simulink model "LKAS_AutoSave_DF_20220221_1634"  (R2018b)
(part 2 of 20)

  | T_p_kPa_1_1_u8.SlopeAdjustmentFactor = 1;
  | T_p_kPa_1_1_u8.Bias = 0;
  | T_p_kPa_1_1_u8.DataTypeOverride = 'Inherit';
  | T_p_kPa_1_1_u8.IsAlias = true;
  | 
  | T_p_kPa_256_1_u16 = Simulink.NumericType;
  | T_p_kPa_256_1_u16.Description = 'kPa (kiloPascals  (kPa))';
  | if (tmpVer > 7.11)
  | 	T_p_kPa_256_1_u16.DataScope = 'Auto';
  | end
  | T_p_kPa_256_1_u16.HeaderFile = 'Rte_Type.h';
  | T_p_kPa_256_1_u16.DataTypeMode = 'Fixed-point: slope and bias scaling';
  | T_p_kPa_256_1_u16.SignednessBool = false;
  | T_p_kPa_256_1_u16.WordLength = 16;
  | T_p_kPa_256_1_u16.FixedExponent = -8;
  | T_p_kPa_256_1_u16.SlopeAdjustmentFactor = 1;
  | T_p_kPa_256_1_u16.Bias = 0;
  | T_p_kPa_256_1_u16.DataTypeOverride = 'Inherit';
  | T_p_kPa_256_1_u16.IsAlias = true;
  | 
  | T_p_kPa_32_1_u16 = Simulink.NumericType;
  | T_p_kPa_32_1_u16.Description = 'kPa (kiloPascals  (kPa))';
  | if (tmpVer > 7.11)
  | 	T_p_kPa_32_1_u16.DataScope = 'Auto';
  | end
  | T_p_kPa_32_1_u16.HeaderFile = 'Rte_Type.h';
  | T_p_kPa_32_1_u16.DataTypeMode = 'Fixed-point: slope and bias scaling';
  | T_p_kPa_32_1_u16.SignednessBool = false;
  | T_p_kPa_32_1_u16.WordLength = 16;
  | T_p_kPa_32_1_u16.FixedExponent = -5;
  | T_p_kPa_32_1_u16.SlopeAdjustmentFactor = 1;
  | T_p_kPa_32_1_u16.Bias = 0;
  | T_p_kPa_32_1_u16.DataTypeOverride = 'Inherit';
  | T_p_kPa_32_1_u16.IsAlias = true;
  | 
  | T_p_kPa_64_1_s16 = Simulink.NumericType;
  | T_p_kPa_64_1_s16.Description = 'kPa (kiloPascals  (kPa))';
  | if (tmpVer > 7.11)
  | 	T_p_kPa_64_1_s16.DataScope = 'Auto';
  | end
  | T_p_kPa_64_1_s16.HeaderFile = 'Rte_Type.h';
  | T_p_kPa_64_1_s16.DataTypeMode = 'Fixed-point: slope and bias scaling';
  | T_p_kPa_64_1_s16.SignednessBool = true;
  | T_p_kPa_64_1_s16.WordLength = 16;
  | T_p_kPa_64_1_s16.FixedExponent = -6;
  | T_p_kPa_64_1_s16.SlopeAdjustmentFactor = 1;
  | T_p_kPa_64_1_s16.Bias = 0;
  | T_p_kPa_64_1_s16.DataTypeOverride = 'Inherit';
  | T_p_kPa_64_1_s16.IsAlias = true;
  | 
  | T_p_kPa_Float32 = Simulink.NumericType;
  | T_p_kPa_Float32.Description = 'kPa (kiloPascals  (kPa))';
  | if (tmpVer > 7.11)
  | 	T_p_kPa_Float32.DataScope = 'Auto';
  | end
  | T_p_kPa_Float32.HeaderFile = 'Rte_Type.h';
  | T_p_kPa_Float32.DataTypeMode = 'Single';
  | T_p_kPa_Float32.SignednessBool = true;
  | T_p_kPa_Float32.WordLength = 32;
  | T_p_kPa_Float32.FixedExponent = 0;
  | T_p_kPa_Float32.SlopeAdjustmentFactor = 1;
  | T_p_kPa_Float32.Bias = 0;
  | T_p_kPa_Float32.DataTypeOverride = 'Inherit';
  | T_p_kPa_Float32.IsAlias = true;
  | 
  | T_phi_deg_100_1_s16 = Simulink.NumericType;
  | T_phi_deg_100_1_s16.Description = 'deg (degrees (deg))';
  | if (tmpVer > 7.11)
  | 	T_phi_deg_100_1_s16.DataScope = 'Auto';
  | end
  | T_phi_deg_100_1_s16.HeaderFile = 'Rte_Type.h';
  | T_phi_deg_100_1_s16.DataTypeMode = ['Fixed-point: slope and bias scalin' ...
  |                                     'g'];
  | T_phi_deg_100_1_s16.SignednessBool = true;
  | T_phi_deg_100_1_s16.WordLength = 16;
  | T_phi_deg_100_1_s16.FixedExponent = -7;
  | T_phi_deg_100_1_s16.SlopeAdjustmentFactor = 1.28;
  | T_phi_deg_100_1_s16.Bias = 0;
  | T_phi_deg_100_1_s16.DataTypeOverride = 'Inherit';
  | T_phi_deg_100_1_s16.IsAlias = true;
  | 
  | T_phi_deg_1024_1_s16 = Simulink.NumericType;
  | T_phi_deg_1024_1_s16.Description = 'deg (degrees (deg))';
  | if (tmpVer > 7.11)
  | 	T_phi_deg_1024_1_s16.DataScope = 'Auto';
  | end
  | T_phi_deg_1024_1_s16.HeaderFile = 'Rte_Type.h';
  | T_phi_deg_1024_1_s16.DataTypeMode = ...
  |   'Fixed-point: slope and bias scaling';
  | T_phi_deg_1024_1_s16.SignednessBool = true;
  | T_phi_deg_1024_1_s16.WordLength = 16;
  | T_phi_deg_1024_1_s16.FixedExponent = -10;
  | T_phi_deg_1024_1_s16.SlopeAdjustmentFactor = 1;
  | T_phi_deg_1024_1_s16.Bias = 0;
  | T_phi_deg_1024_1_s16.DataTypeOverride = 'Inherit';
  | T_phi_deg_1024_1_s16.IsAlias = true;
  | 
  | T_phi_deg_128_1_s16 = Simulink.NumericType;
  | T_phi_deg_128_1_s16.Description = 'deg (degrees (deg))';
  | if (tmpVer > 7.11)
  | 	T_phi_deg_128_1_s16.DataScope = 'Auto';
  | end
  | T_phi_deg_128_1_s16.HeaderFile = 'Rte_Type.h';
  | T_phi_deg_128_1_s16.DataTypeMode = ['Fixed-point: slope and bias scalin' ...
  |                                     'g'];
  | T_phi_deg_128_1_s16.SignednessBool = true;
  | T_phi_deg_128_1_s16.WordLength = 16;
  | T_phi_deg_128_1_s16.FixedExponent = -7;
  | T_phi_deg_128_1_s16.SlopeAdjustmentFactor = 1;
  | T_phi_deg_128_1_s16.Bias = 0;
  | T_phi_deg_128_1_s16.DataTypeOverride = 'Inherit';
  | T_phi_deg_128_1_s16.IsAlias = true;
  | 
  | T_phi_deg_1_1_u8 = Simulink.NumericType;
  | T_phi_deg_1_1_u8.Description = 'deg (degrees (deg))';
  | if (tmpVer > 7.11)
  | 	T_phi_deg_1_1_u8.DataScope = 'Auto';
  | end
  | T_phi_deg_1_1_u8.HeaderFile = 'Rte_Type.h';
  | T_phi_deg_1_1_u8.DataTypeMode = 'Fixed-point: slope and bias scaling';
  | T_phi_deg_1_1_u8.SignednessBool = false;
  | T_phi_deg_1_1_u8.WordLength = 8;
  | T_phi_deg_1_1_u8.FixedExponent = 0;
  | T_phi_deg_1_1_u8.SlopeAdjustmentFactor = 1;
  | T_phi_deg_1_1_u8.Bias = 0;
  | T_phi_deg_1_1_u8.DataTypeOverride = 'Inherit';
  | T_phi_deg_1_1_u8.IsAlias = true;
  | 
  | T_phi_deg_256_1_s16 = Simulink.NumericType;
  | T_phi_deg_256_1_s16.Description = 'deg (degrees (deg))';
  | if (tmpVer > 7.11)
  | 	T_phi_deg_256_1_s16.DataScope = 'Auto';
  | end
  | T_phi_deg_256_1_s16.HeaderFile = 'Rte_Type.h';
  | T_phi_deg_256_1_s16.DataTypeMode = ['Fixed-point: slope and bias scalin' ...
  |                                     'g'];
  | T_phi_deg_256_1_s16.SignednessBool = true;
  | T_phi_deg_256_1_s16.WordLength = 16;
  | T_phi_deg_256_1_s16.FixedExponent = -8;
  | T_phi_deg_256_1_s16.SlopeAdjustmentFactor = 1;
  | T_phi_deg_256_1_s16.Bias = 0;
  | T_phi_deg_256_1_s16.DataTypeOverride = 'Inherit';
  | T_phi_deg_256_1_s16.IsAlias = true;
  | 
  | T_phi_deg_2_1_s8 = Simulink.NumericType;
  | T_phi_deg_2_1_s8.Description = 'deg (degrees (deg))';
  | if (tmpVer > 7.11)
  | 	T_phi_deg_2_1_s8.DataScope = 'Auto';
  | end
  | T_phi_deg_2_1_s8.HeaderFile = 'Rte_Type.h';
  | T_phi_deg_2_1_s8.DataTypeMode = 'Fixed-point: slope and bias scaling';
  | T_phi_deg_2_1_s8.SignednessBool = true;
  | T_phi_deg_2_1_s8.WordLength = 8;
  | T_phi_deg_2_1_s8.FixedExponent = -1;
  | T_phi_deg_2_1_s8.SlopeAdjustmentFactor = 1;
  | T_phi_deg_2_1_s8.Bias = 0;
  | T_phi_deg_2_1_s8.DataTypeOverride = 'Inherit';
  | T_phi_deg_2_1_s8.IsAlias = true;
  | 
  | T_phi_deg_32_1_s16 = Simulink.NumericType;
  | T_phi_deg_32_1_s16.Description = 'deg (degrees (deg))';
  | if (tmpVer > 7.11)
  | 	T_phi_deg_32_1_s16.DataScope = 'Auto';
  | end
  | T_phi_deg_32_1_s16.HeaderFile = 'Rte_Type.h';
  | T_phi_deg_32_1_s16.DataTypeMode = 'Fixed-point: slope and bias scaling';
  | T_phi_deg_32_1_s16.SignednessBool = true;
  | T_phi_deg_32_1_s16.WordLength = 16;
  | T_phi_deg_32_1_s16.FixedExponent = -5;
  | T_phi_deg_32_1_s16.SlopeAdjustmentFactor = 1;
  | T_phi_deg_32_1_s16.Bias = 0;
  | T_phi_deg_32_1_s16.DataTypeOverride = 'Inherit';
  | T_phi_deg_32_1_s16.IsAlias = true;
  | 
  | T_phi_deg_512_6_s32 = Simulink.NumericType;
  | T_phi_deg_512_6_s32.Description = 'deg (degrees (deg))';
  | if (tmpVer > 7.11)
  | 	T_phi_deg_512_6_s32.DataScope = 'Auto';
  | end
  | T_phi_deg_512_6_s32.HeaderFile = 'Rte_Type.h';
  | T_phi_deg_512_6_s32.DataTypeMode = ['Fixed-point: slope and bias scalin' ...
  |                                     'g'];
  | T_phi_deg_512_6_s32.SignednessBool = true;
  | T_phi_deg_512_6_s32.WordLength = 32;
  | T_phi_deg_512_6_s32.FixedExponent = -7;
  | T_phi_deg_512_6_s32.SlopeAdjustmentFactor = 1.5;
  | T_phi_deg_512_6_s32.Bias = 0;
  | T_phi_deg_512_6_s32.DataTypeOverride = 'Inherit';
  | T_phi_deg_512_6_s32.IsAlias = true;
  | 
  | T_phi_deg_Float32 = Simulink.NumericType;
  | T_phi_deg_Float32.Description = 'deg (degrees (deg))';
  | if (tmpVer > 7.11)
  | 	T_phi_deg_Float32.DataScope = 'Auto';
  | end
  | T_phi_deg_Float32.HeaderFile = 'Rte_Type.h';
  | T_phi_deg_Float32.DataTypeMode = 'Single';
  | T_phi_deg_Float32.SignednessBool = true;
  | T_phi_deg_Float32.WordLength = 32;
  | T_phi_deg_Float32.FixedExponent = 0;
  | T_phi_deg_Float32.SlopeAdjustmentFactor = 1;
  | T_phi_deg_Float32.Bias = 0;
  | T_phi_deg_Float32.DataTypeOverride = 'Inherit';
  | T_phi_deg_Float32.IsAlias = true;
  | 
  | T_phi_rad_2048_1_s16 = Simulink.NumericType;
  | T_phi_rad_2048_1_s16.Description = 'rad (radians  (rad))';
  | if (tmpVer > 7.11)
  | 	T_phi_rad_2048_1_s16.DataScope = 'Auto';
  | end
  | T_phi_rad_2048_1_s16.HeaderFile = 'Rte_Type.h';
  | T_phi_rad_2048_1_s16.DataTypeMode = ...
  |   'Fixed-point: slope and bias scaling';
  | T_phi_rad_2048_1_s16.SignednessBool = true;
  | T_phi_rad_2048_1_s16.WordLength = 16;
  | T_phi_rad_2048_1_s16.FixedExponent = -11;
  | T_phi_rad_2048_1_s16.SlopeAdjustmentFactor = 1;
  | T_phi_rad_2048_1_s16.Bias = 0;
  | T_phi_rad_2048_1_s16.DataTypeOverride = 'Inherit';
  | T_phi_rad_2048_1_s16.IsAlias = true;
  | 
  | T_phi_rad_Float32 = Simulink.NumericType;
  | T_phi_rad_Float32.Description = 'rad (radians  (rad))';
  | if (tmpVer > 7.11)
  | 	T_phi_rad_Float32.DataScope = 'Auto';
  | end
  | T_phi_rad_Float32.HeaderFile = 'Rte_Type.h';
  | T_phi_rad_Float32.DataTypeMode = 'Single';
  | T_phi_rad_Float32.SignednessBool = true;
  | T_phi_rad_Float32.WordLength = 32;
  | T_phi_rad_Float32.FixedExponent = 0;
  | T_phi_rad_Float32.SlopeAdjustmentFactor = 1;
  | T_phi_rad_Float32.Bias = 0;
  | T_phi_rad_Float32.DataTypeOverride = 'Inherit';
  | T_phi_rad_Float32.IsAlias = true;
  | 
  | T_r_NA_1024_1_s16 = Simulink.NumericType;
  | T_r_NA_1024_1_s16.Description = 'NA (none)';
  | if (tmpVer > 7.11)
  | 	T_r_NA_1024_1_s16.DataScope = 'Auto';
  | end
  | T_r_NA_1024_1_s16.HeaderFile = 'Rte_Type.h';
  | T_r_NA_1024_1_s16.DataTypeMode = 'Fixed-point: slope and bias scaling';
  | T_r_NA_1024_1_s16.SignednessBool = true;
  | T_r_NA_1024_1_s16.WordLength = 16;
  | T_r_NA_1024_1_s16.FixedExponent = -10;
  | T_r_NA_1024_1_s16.SlopeAdjustmentFactor = 1;
  | T_r_NA_1024_1_s16.Bias = 0;
  | T_r_NA_1024_1_s16.DataTypeOverride = 'Inherit';
  | T_r_NA_1024_1_s16.IsAlias = true;
  | 
  | T_r_NA_1024_1_u16 = Simulink.NumericType;
  | T_r_NA_1024_1_u16.Description = 'NA (none)';
  | if (tmpVer > 7.11)
  | 	T_r_NA_1024_1_u16.DataScope = 'Auto';
  | end
  | T_r_NA_1024_1_u16.HeaderFile = 'Rte_Type.h';
  | T_r_NA_1024_1_u16.DataTypeMode = 'Fixed-point: slope and bias scaling';
  | T_r_NA_1024_1_u16.SignednessBool = false;
  | T_r_NA_1024_1_u16.WordLength = 16;
  | T_r_NA_1024_1_u16.FixedExponent = -10;
  | T_r_NA_1024_1_u16.SlopeAdjustmentFactor = 1;
  | T_r_NA_1024_1_u16.Bias = 0;
  | T_r_NA_1024_1_u16.DataTypeOverride = 'Inherit';
  | T_r_NA_1024_1_u16.IsAlias = true;
  | 
  | T_r_NA_16384_1_s16 = Simulink.NumericType;
  | T_r_NA_16384_1_s16.Description = 'NA (none)';
  | if (tmpVer > 7.11)
  | 	T_r_NA_16384_1_s16.DataScope = 'Auto';
  | end
  | T_r_NA_16384_1_s16.HeaderFile = 'Rte_Type.h';
  | T_r_NA_16384_1_s16.DataTypeMode = 'Fixed-point: slope and bias scaling';
  | T_r_NA_16384_1_s16.SignednessBool = true;
  | T_r_NA_16384_1_s16.WordLength = 16;
  | T_r_NA_16384_1_s16.FixedExponent = -14;
  | T_r_NA_16384_1_s16.SlopeAdjustmentFactor = 1;
  | T_r_NA_16384_1_s16.Bias = 0;
  | T_r_NA_16384_1_s16.DataTypeOverride = 'Inherit';
  | T_r_NA_16384_1_s16.IsAlias = true;
  | 
  | T_r_NA_16_1_s16 = Simulink.NumericType;
  | T_r_NA_16_1_s16.Description = 'NA (none)';
  | if (tmpVer > 7.11)
  | 	T_r_NA_16_1_s16.DataScope = 'Auto';
  | end
  | T_r_NA_16_1_s16.HeaderFile = 'Rte_Type.h';
  | T_r_NA_16_1_s16.DataTypeMode = 'Fixed-point: slope and bias scaling';
  | T_r_NA_16_1_s16.SignednessBool = true;
  | T_r_NA_16_1_s16.WordLength = 16;
  | T_r_NA_16_1_s16.FixedExponent = -4;
  | T_r_NA_16_1_s16.SlopeAdjustmentFactor = 1;
  | T_r_NA_16_1_s16.Bias = 0;
  | T_r_NA_16_1_s16.DataTypeOverride = 'Inherit';
  | T_r_NA_16_1_s16.IsAlias = true;
  | 
  | T_r_NA_256_1_s8 = Simulink.NumericType;
  | T_r_NA_256_1_s8.Description = 'NA (none)';
  | if (tmpVer > 7.11)
  | 	T_r_NA_256_1_s8.DataScope = 'Auto';
  | end
  | T_r_NA_256_1_s8.HeaderFile = 'Rte_Type.h';
  | T_r_NA_256_1_s8.DataTypeMode = 'Fixed-point: slope and bias scaling';
  | T_r_NA_256_1_s8.SignednessBool = true;
  | T_r_NA_256_1_s8.WordLength = 8;
  | T_r_NA_256_1_s8.FixedExponent = -8;
  | T_r_NA_256_1_s8.SlopeAdjustmentFactor = 1;
  | T_r_NA_256_1_s8.Bias = 0;
  | T_r_NA_256_1_s8.DataTypeOverride = 'Inherit';
  | T_r_NA_256_1_s8.IsAlias = true;
  | 
  | T_r_NA_256_1_u16 = Simulink.NumericType;
  | T_r_NA_256_1_u16.Description = 'NA (none)';
  | if (tmpVer > 7.11)
  | 	T_r_NA_256_1_u16.DataScope = 'Auto';
  | end
  | T_r_NA_256_1_u16.HeaderFile = 'Rte_Type.h';
  | T_r_NA_256_1_u16.DataTypeMode = 'Fixed-point: slope and bias scaling';
  | T_r_NA_256_1_u16.SignednessBool = false;
  | T_r_NA_256_1_u16.WordLength = 16;
  | T_r_NA_256_1_u16.FixedExponent = -8;
  | T_r_NA_256_1_u16.SlopeAdjustmentFactor = 1;
  | T_r_NA_256_1_u16.Bias = 0;
  | T_r_NA_256_1_u16.DataTypeOverride = 'Inherit';
  | T_r_NA_256_1_u16.IsAlias = true;
  | 
  | T_r_NA_32768_1_u16 = Simulink.NumericType;
  | T_r_NA_32768_1_u16.Description = 'NA (none)';
  | if (tmpVer > 7.11)
  | 	T_r_NA_32768_1_u16.DataScope = 'Auto';
  | end
  | T_r_NA_32768_1_u16.HeaderFile = 'Rte_Type.h';
  | T_r_NA_32768_1_u16.DataTypeMode = 'Fixed-point: slope and bias scaling';
  | T_r_NA_32768_1_u16.SignednessBool = false;
  | T_r_NA_32768_1_u16.WordLength = 16;
  | T_r_NA_32768_1_u16.FixedExponent = -15;
  | T_r_NA_32768_1_u16.SlopeAdjustmentFactor = 1;
  | T_r_NA_32768_1_u16.Bias = 0;
  | T_r_NA_32768_1_u16.DataTypeOverride = 'Inherit';
  | T_r_NA_32768_1_u16.IsAlias = true;
  | 
  | T_r_NA_32_1_u16 = Simulink.NumericType;
  | T_r_NA_32_1_u16.Description = 'NA (none)';
  | if (tmpVer > 7.11)
  | 	T_r_NA_32_1_u16.DataScope = 'Auto';
  | end
  | T_r_NA_32_1_u16.HeaderFile = 'Rte_Type.h';
  | T_r_NA_32_1_u16.DataTypeMode = 'Fixed-point: slope and bias scaling';
  | T_r_NA_32_1_u16.SignednessBool = false;
  | T_r_NA_32_1_u16.WordLength = 16;
  | T_r_NA_32_1_u16.FixedExponent = -5;
  | T_r_NA_32_1_u16.SlopeAdjustmentFactor = 1;
  | T_r_NA_32_1_u16.Bias = 0;
  | T_r_NA_32_1_u16.DataTypeOverride = 'Inherit';
  | T_r_NA_32_1_u16.IsAlias = true;
  | 
  | T_r_NA_4096_1_s16 = Simulink.NumericType;
  | T_r_NA_4096_1_s16.Description = 'NA (none)';
  | if (tmpVer > 7.11)
  | 	T_r_NA_4096_1_s16.DataScope = 'Auto';
  | end
  | T_r_NA_4096_1_s16.HeaderFile = 'Rte_Type.h';
  | T_r_NA_4096_1_s16.DataTypeMode = 'Fixed-point: slope and bias scaling';
  | T_r_NA_4096_1_s16.SignednessBool = true;
  | T_r_NA_4096_1_s16.WordLength = 16;
  | T_r_NA_4096_1_s16.FixedExponent = -12;
  | T_r_NA_4096_1_s16.SlopeAdjustmentFactor = 1;
  | T_r_NA_4096_1_s16.Bias = 0;
  | T_r_NA_4096_1_s16.DataTypeOverride = 'Inherit';
  | T_r_NA_4096_1_s16.IsAlias = true;
  | 
  | T_r_NA_65535_2_u16 = Simulink.NumericType;
  | T_r_NA_65535_2_u16.Description = 'NA (none)';
  | if (tmpVer > 7.11)
  | 	T_r_NA_65535_2_u16.DataScope = 'Auto';
  | end
  | T_r_NA_65535_2_u16.HeaderFile = 'Rte_Type.h';
  | T_r_NA_65535_2_u16.DataTypeMode = 'Fixed-point: slope and bias scaling';
  | T_r_NA_65535_2_u16.SignednessBool = false;
  | T_r_NA_65535_2_u16.WordLength = 16;
  | T_r_NA_65535_2_u16.FixedExponent = -15;
  | T_r_NA_65535_2_u16.SlopeAdjustmentFactor = 1.0000152590218967;
  | T_r_NA_65535_2_u16.Bias = 0;
  | T_r_NA_65535_2_u16.DataTypeOverride = 'Inherit';
  | T_r_NA_65535_2_u16.IsAlias = true;
  | 
  | T_r_NA_8192_1_u16 = Simulink.NumericType;
  | T_r_NA_8192_1_u16.Description = 'NA (none)';
  | if (tmpVer > 7.11)
  | 	T_r_NA_8192_1_u16.DataScope = 'Auto';
  | end
  | T_r_NA_8192_1_u16.HeaderFile = 'Rte_Type.h';
  | T_r_NA_8192_1_u16.DataTypeMode = 'Fixed-point: slope and bias scaling';
  | T_r_NA_8192_1_u16.SignednessBool = false;
  | T_r_NA_8192_1_u16.WordLength = 16;
  | T_r_NA_8192_1_u16.FixedExponent = -13;
  | T_r_NA_8192_1_u16.SlopeAdjustmentFactor = 1;
  | T_r_NA_8192_1_u16.Bias = 0;
  | T_r_NA_8192_1_u16.DataTypeOverride = 'Inherit';
  | T_r_NA_8192_1_u16.IsAlias = true;
  | 
  | T_r_NA_Float32 = Simulink.NumericType;
  | T_r_NA_Float32.Description = 'NA (none)';
  | if (tmpVer > 7.11)
  | 	T_r_NA_Float32.DataScope = 'Auto';
  | end
  | T_r_NA_Float32.HeaderFile = 'Rte_Type.h';
  | T_r_NA_Float32.DataTypeMode = 'Single';
  | T_r_NA_Float32.SignednessBool = true;
  | T_r_NA_Float32.WordLength = 32;
  | T_r_NA_Float32.FixedExponent = 0;
  | T_r_NA_Float32.SlopeAdjustmentFactor = 1;
  | T_r_NA_Float32.Bias = 0;
  | T_r_NA_Float32.DataTypeOverride = 'Inherit';
  | T_r_NA_Float32.IsAlias = true;
  | 
  | T_rho_gpl_8192_1_s16 = Simulink.NumericType;
  | T_rho_gpl_8192_1_s16.Description = 'gpl (grams / liter  (g/l))';
  | if (tmpVer > 7.11)
  | 	T_rho_gpl_8192_1_s16.DataScope = 'Auto';
  | end
  | T_rho_gpl_8192_1_s16.HeaderFile = 'Rte_Type.h';
  | T_rho_gpl_8192_1_s16.DataTypeMode = ...
  |   'Fixed-point: slope and bias scaling';
  | T_rho_gpl_8192_1_s16.SignednessBool = true;
  | T_rho_gpl_8192_1_s16.WordLength = 16;
  | T_rho_gpl_8192_1_s16.FixedExponent = -13;
  | T_rho_gpl_8192_1_s16.SlopeAdjustmentFactor = 1;
  | T_rho_gpl_8192_1_s16.Bias = 0;
  | T_rho_gpl_8192_1_s16.DataTypeOverride = 'Inherit';
  | T_rho_gpl_8192_1_s16.IsAlias = true;
  | 
  | T_rho_gpl_Float32 = Simulink.NumericType;
  | T_rho_gpl_Float32.Description = 'gpl (grams / liter  (g/l))';
  | if (tmpVer > 7.11)
  | 	T_rho_gpl_Float32.DataScope = 'Auto';
  | end
  | T_rho_gpl_Float32.HeaderFile = 'Rte_Type.h';
  | T_rho_gpl_Float32.DataTypeMode = 'Single';
  | T_rho_gpl_Float32.SignednessBool = true;
  | T_rho_gpl_Float32.WordLength = 32;
  | T_rho_gpl_Float32.FixedExponent = 0;
  | T_rho_gpl_Float32.SlopeAdjustmentFactor = 1;
  | T_rho_gpl_Float32.Bias = 0;
  | T_rho_gpl_Float32.DataTypeOverride = 'Inherit';
  | T_rho_gpl_Float32.IsAlias = true;
  | 
  | T_rho_kgpm3_16_1_s16 = Simulink.NumericType;
  | T_rho_kgpm3_16_1_s16.Description = ['kgpm3 (kilograms / cubic meter  (k' ...
  |                                     'g/m3))'];
  | if (tmpVer > 7.11)
  | 	T_rho_kgpm3_16_1_s16.DataScope = 'Auto';
  | end
  | T_rho_kgpm3_16_1_s16.HeaderFile = 'Rte_Type.h';
  | T_rho_kgpm3_16_1_s16.DataTypeMode = ...
  |   'Fixed-point: slope and bias scaling';
  | T_rho_kgpm3_16_1_s16.SignednessBool = true;
  | T_rho_kgpm3_16_1_s16.WordLength = 16;
  | T_rho_kgpm3_16_1_s16.FixedExponent = -4;
  | T_rho_kgpm3_16_1_s16.SlopeAdjustmentFactor = 1;
  | T_rho_kgpm3_16_1_s16.Bias = 0;
  | T_rho_kgpm3_16_1_s16.DataTypeOverride = 'Inherit';
  | T_rho_kgpm3_16_1_s16.IsAlias = true;
  | 
  | T_rho_kgpm3_Float32 = Simulink.NumericType;
  | T_rho_kgpm3_Float32.Description = ['kgpm3 (kilograms / cubic meter  (kg' ...
  |                                    '/m3))'];
  | if (tmpVer > 7.11)
  | 	T_rho_kgpm3_Float32.DataScope = 'Auto';
  | end
  | T_rho_kgpm3_Float32.HeaderFile = 'Rte_Type.h';
  | T_rho_kgpm3_Float32.DataTypeMode = 'Single';
  | T_rho_kgpm3_Float32.SignednessBool = true;
  | T_rho_kgpm3_Float32.WordLength = 32;
  | T_rho_kgpm3_Float32.FixedExponent = 0;
  | T_rho_kgpm3_Float32.SlopeAdjustmentFactor = 1;
  | T_rho_kgpm3_Float32.Bias = 0;
  | T_rho_kgpm3_Float32.DataTypeOverride = 'Inherit';
  | T_rho_kgpm3_Float32.IsAlias = true;
  | 
  | T_rho_mgpl_1_1_s16 = Simulink.NumericType;
  | T_rho_mgpl_1_1_s16.Description = 'mgpl (milligrams / liter  (mg/l))';
  | if (tmpVer > 7.11)
  | 	T_rho_mgpl_1_1_s16.DataScope = 'Auto';
  | end
  | T_rho_mgpl_1_1_s16.HeaderFile = 'Rte_Type.h';
  | T_rho_mgpl_1_1_s16.DataTypeMode = 'Fixed-point: slope and bias scaling';
  | T_rho_mgpl_1_1_s16.SignednessBool = true;
  | T_rho_mgpl_1_1_s16.WordLength = 16;
  | T_rho_mgpl_1_1_s16.FixedExponent = 0;
  | T_rho_mgpl_1_1_s16.SlopeAdjustmentFactor = 1;
  | T_rho_mgpl_1_1_s16.Bias = 0;
  | T_rho_mgpl_1_1_s16.DataTypeOverride = 'Inherit';
  | T_rho_mgpl_1_1_s16.IsAlias = true;
  | 
  | T_rho_mgpl_64_1_s16 = Simulink.NumericType;
  | T_rho_mgpl_64_1_s16.Description = 'mgpl (milligrams / liter  (mg/l))';
  | if (tmpVer > 7.11)
  | 	T_rho_mgpl_64_1_s16.DataScope = 'Auto';
  | end
  | T_rho_mgpl_64_1_s16.HeaderFile = 'Rte_Type.h';
  | T_rho_mgpl_64_1_s16.DataTypeMode = ['Fixed-point: slope and bias scalin' ...
  |                                     'g'];
  | T_rho_mgpl_64_1_s16.SignednessBool = true;
  | T_rho_mgpl_64_1_s16.WordLength = 16;
  | T_rho_mgpl_64_1_s16.FixedExponent = -6;
  | T_rho_mgpl_64_1_s16.SlopeAdjustmentFactor = 1;
  | T_rho_mgpl_64_1_s16.Bias = 0;
  | T_rho_mgpl_64_1_s16.DataTypeOverride = 'Inherit';
  | T_rho_mgpl_64_1_s16.IsAlias = true;
  | 
  | T_rho_mgpl_Float32 = Simulink.NumericType;
  | T_rho_mgpl_Float32.Description = 'mgpl (milligrams / liter  (mg/l))';
  | if (tmpVer > 7.11)
  | 	T_rho_mgpl_Float32.DataScope = 'Auto';
  | end
  | T_rho_mgpl_Float32.HeaderFile = 'Rte_Type.h';
  | T_rho_mgpl_Float32.DataTypeMode = 'Single';
  | T_rho_mgpl_Float32.SignednessBool = true;
  | T_rho_mgpl_Float32.WordLength = 32;
  | T_rho_mgpl_Float32.FixedExponent = 0;
  | T_rho_mgpl_Float32.SlopeAdjustmentFactor = 1;
  | T_rho_mgpl_Float32.Bias = 0;
  | T_rho_mgpl_Float32.DataTypeOverride = 'Inherit';
  | T_rho_mgpl_Float32.IsAlias = true;
  | 
  | T_t_hour_1_1_s16 = Simulink.NumericType;
  | T_t_hour_1_1_s16.Description = 'h (hour  (h))';
  | if (tmpVer > 7.11)
  | 	T_t_hour_1_1_s16.DataScope = 'Auto';
  | end
  | T_t_hour_1_1_s16.HeaderFile = 'Rte_Type.h';
  | T_t_hour_1_1_s16.DataTypeMode = 'Fixed-point: slope and bias scaling';
  | T_t_hour_1_1_s16.SignednessBool = true;
  | T_t_hour_1_1_s16.WordLength = 16;
  | T_t_hour_1_1_s16.FixedExponent = 0;
  | T_t_hour_1_1_s16.SlopeAdjustmentFactor = 1;
  | T_t_hour_1_1_s16.Bias = 0;
  | T_t_hour_1_1_s16.DataTypeOverride = 'Inherit';
  | T_t_hour_1_1_s16.IsAlias = true;
  | 
  | T_t_hour_Float32 = Simulink.NumericType;
  | T_t_hour_Float32.Description = 'h (hour  (h))';
  | if (tmpVer > 7.11)
  | 	T_t_hour_Float32.DataScope = 'Auto';
  | end
  | T_t_hour_Float32.HeaderFile = 'Rte_Type.h';
  | T_t_hour_Float32.DataTypeMode = 'Single';
  | T_t_hour_Float32.SignednessBool = true;
  | T_t_hour_Float32.WordLength = 32;
  | T_t_hour_Float32.FixedExponent = 0;
  | T_t_hour_Float32.SlopeAdjustmentFactor = 1;
  | T_t_hour_Float32.Bias = 0;
  | T_t_hour_Float32.DataTypeOverride = 'Inherit';
  | T_t_hour_Float32.IsAlias = true;
  | 
  | T_t_m_1_1_u16 = Simulink.NumericType;
  | T_t_m_1_1_u16.Description = 'm (minutes  (m))';
  | if (tmpVer > 7.11)
  | 	T_t_m_1_1_u16.DataScope = 'Auto';
  | end
  | T_t_m_1_1_u16.HeaderFile = 'Rte_Type.h';
  | T_t_m_1_1_u16.DataTypeMode = 'Fixed-point: slope and bias scaling';
  | T_t_m_1_1_u16.SignednessBool = false;
  | T_t_m_1_1_u16.WordLength = 16;
  | T_t_m_1_1_u16.FixedExponent = 0;
  | T_t_m_1_1_u16.SlopeAdjustmentFactor = 1;
  | T_t_m_1_1_u16.Bias = 0;
  | T_t_m_1_1_u16.DataTypeOverride = 'Inherit';
  | T_t_m_1_1_u16.IsAlias = true;
  | 
  | T_t_m_Float32 = Simulink.NumericType;
  | T_t_m_Float32.Description = 'm (minutes  (m))';
  | if (tmpVer > 7.11)
  | 	T_t_m_Float32.DataScope = 'Auto';
  | end
  | T_t_m_Float32.HeaderFile = 'Rte_Type.h';
  | T_t_m_Float32.DataTypeMode = 'Single';
  | T_t_m_Float32.SignednessBool = true;
  | T_t_m_Float32.WordLength = 32;
  | T_t_m_Float32.FixedExponent = 0;
  | T_t_m_Float32.SlopeAdjustmentFactor = 1;
  | T_t_m_Float32.Bias = 0;
  | T_t_m_Float32.DataTypeOverride = 'Inherit';
  | T_t_m_Float32.IsAlias = true;
  | 
  | T_t_ms_1_1_s16 = Simulink.NumericType;
  | T_t_ms_1_1_s16.Description = 'ms (milliseconds  (ms))';
  | if (tmpVer > 7.11)
  | 	T_t_ms_1_1_s16.DataScope = 'Auto';
  | end
  | T_t_ms_1_1_s16.HeaderFile = 'Rte_Type.h';
  | T_t_ms_1_1_s16.DataTypeMode = 'Fixed-point: slope and bias scaling';
  | T_t_ms_1_1_s16.SignednessBool = true;
  | T_t_ms_1_1_s16.WordLength = 16;
  | T_t_ms_1_1_s16.FixedExponent = 0;
  | T_t_ms_1_1_s16.SlopeAdjustmentFactor = 1;
  | T_t_ms_1_1_s16.Bias = 0;
  | T_t_ms_1_1_s16.DataTypeOverride = 'Inherit';
  | T_t_ms_1_1_s16.IsAlias = true;
  | 
  | T_t_ms_1_1_u16 = Simulink.NumericType;
  | T_t_ms_1_1_u16.Description = 'ms (milliseconds  (ms))';
  | if (tmpVer > 7.11)
  | 	T_t_ms_1_1_u16.DataScope = 'Auto';
  | end
  | T_t_ms_1_1_u16.HeaderFile = 'Rte_Type.h';
  | T_t_ms_1_1_u16.DataTypeMode = 'Fixed-point: slope and bias scaling';
  | T_t_ms_1_1_u16.SignednessBool = false;
  | T_t_ms_1_1_u16.WordLength = 16;
  | T_t_ms_1_1_u16.FixedExponent = 0;
  | T_t_ms_1_1_u16.SlopeAdjustmentFactor = 1;
  | T_t_ms_1_1_u16.Bias = 0;
  | T_t_ms_1_1_u16.DataTypeOverride = 'Inherit';
  | T_t_ms_1_1_u16.IsAlias = true;
  | 
  | T_t_ms_1_1_u32 = Simulink.NumericType;
  | T_t_ms_1_1_u32.Description = 'ms (milliseconds  (ms))';
  | if (tmpVer > 7.11)
  | 	T_t_ms_1_1_u32.DataScope = 'Auto';
  | end
  | T_t_ms_1_1_u32.HeaderFile = 'Rte_Type.h';
  | T_t_ms_1_1_u32.DataTypeMode = 'Fixed-point: slope and bias scaling';
  | T_t_ms_1_1_u32.SignednessBool = false;
  | T_t_ms_1_1_u32.WordLength = 32;
  | T_t_ms_1_1_u32.FixedExponent = 0;
  | T_t_ms_1_1_u32.SlopeAdjustmentFactor = 1;
  | T_t_ms_1_1_u32.Bias = 0;
  | T_t_ms_1_1_u32.DataTypeOverride = 'Inherit';
  | T_t_ms_1_1_u32.IsAlias = true;
  | 
  | T_t_ms_4096_1_s16 = Simulink.NumericType;
  | T_t_ms_4096_1_s16.Description = 'ms (milliseconds  (ms))';
  | if (tmpVer > 7.11)
  | 	T_t_ms_4096_1_s16.DataScope = 'Auto';
  | end
  | T_t_ms_4096_1_s16.HeaderFile = 'Rte_Type.h';
  | T_t_ms_4096_1_s16.DataTypeMode = 'Fixed-point: slope and bias scaling';
  | T_t_ms_4096_1_s16.SignednessBool = true;
  | T_t_ms_4096_1_s16.WordLength = 16;
  | T_t_ms_4096_1_s16.FixedExponent = -12;
  | T_t_ms_4096_1_s16.SlopeAdjustmentFactor = 1;
  | T_t_ms_4096_1_s16.Bias = 0;
  | T_t_ms_4096_1_s16.DataTypeOverride = 'Inherit';
  | T_t_ms_4096_1_s16.IsAlias = true;
  | 
  | T_t_ms_64_1_s16 = Simulink.NumericType;
  | T_t_ms_64_1_s16.Description = 'ms (milliseconds  (ms))';
  | if (tmpVer > 7.11)
  | 	T_t_ms_64_1_s16.DataScope = 'Auto';
  | end
  | T_t_ms_64_1_s16.HeaderFile = 'Rte_Type.h';
  | T_t_ms_64_1_s16.DataTypeMode = 'Fixed-point: slope and bias scaling';
  | T_t_ms_64_1_s16.SignednessBool = true;
  | T_t_ms_64_1_s16.WordLength = 16;
  | T_t_ms_64_1_s16.FixedExponent = -6;
  | T_t_ms_64_1_s16.SlopeAdjustmentFactor = 1;
  | T_t_ms_64_1_s16.Bias = 0;
  | T_t_ms_64_1_s16.DataTypeOverride = 'Inherit';
  | T_t_ms_64_1_s16.IsAlias = true;
  | 
  | T_t_ms_Float32 = Simulink.NumericType;
  | T_t_ms_Float32.Description = 'ms (milliseconds  (ms))';
  | if (tmpVer > 7.11)
  | 	T_t_ms_Float32.DataScope = 'Auto';
  | end
  | T_t_ms_Float32.HeaderFile = 'Rte_Type.h';
  | T_t_ms_Float32.DataTypeMode = 'Single';
  | T_t_ms_Float32.SignednessBool = true;
  | T_t_ms_Float32.WordLength = 32;
  | T_t_ms_Float32.FixedExponent = 0;
  | T_t_ms_Float32.SlopeAdjustmentFactor = 1;
  | T_t_ms_Float32.Bias = 0;
  | T_t_ms_Float32.DataTypeOverride = 'Inherit';
  | T_t_ms_Float32.IsAlias = true;
  | 
  | T_t_s_1000_1_s16 = Simulink.NumericType;
  | T_t_s_1000_1_s16.Description = 's (seconds  (s))';
  | if (tmpVer > 7.11)
  | 	T_t_s_1000_1_s16.DataScope = 'Auto';
  | end
  | T_t_s_1000_1_s16.HeaderFile = 'Rte_Type.h';
  | T_t_s_1000_1_s16.DataTypeMode = 'Fixed-point: slope and bias scaling';
  | T_t_s_1000_1_s16.SignednessBool = true;
  | T_t_s_1000_1_s16.WordLength = 16;
  | T_t_s_1000_1_s16.FixedExponent = -10;
  | T_t_s_1000_1_s16.SlopeAdjustmentFactor = 1.024;
  | T_t_s_1000_1_s16.Bias = 0;
  | T_t_s_1000_1_s16.DataTypeOverride = 'Inherit';
  | T_t_s_1000_1_s16.IsAlias = true;
  | 
  | T_t_s_100_1_s16 = Simulink.NumericType;
  | T_t_s_100_1_s16.Description = 's (seconds  (s))';
  | if (tmpVer > 7.11)
  | 	T_t_s_100_1_s16.DataScope = 'Auto';
  | end
  | T_t_s_100_1_s16.HeaderFile = 'Rte_Type.h';
  | T_t_s_100_1_s16.DataTypeMode = 'Fixed-point: slope and bias scaling';
  | T_t_s_100_1_s16.SignednessBool = true;
  | T_t_s_100_1_s16.WordLength = 16;
  | T_t_s_100_1_s16.FixedExponent = -7;
  | T_t_s_100_1_s16.SlopeAdjustmentFactor = 1.28;
  | T_t_s_100_1_s16.Bias = 0;
  | T_t_s_100_1_s16.DataTypeOverride = 'Inherit';
  | T_t_s_100_1_s16.IsAlias = true;
  | 
  | T_t_s_10_1_s16 = Simulink.NumericType;
  | T_t_s_10_1_s16.Description = 's (seconds  (s))';
  | if (tmpVer > 7.11)
  | 	T_t_s_10_1_s16.DataScope = 'Auto';
  | end
  | T_t_s_10_1_s16.HeaderFile = 'Rte_Type.h';
  | T_t_s_10_1_s16.DataTypeMode = 'Fixed-point: slope and bias scaling';
  | T_t_s_10_1_s16.SignednessBool = true;
  | T_t_s_10_1_s16.WordLength = 16;
  | T_t_s_10_1_s16.FixedExponent = -4;
  | T_t_s_10_1_s16.SlopeAdjustmentFactor = 1.6;
  | T_t_s_10_1_s16.Bias = 0;
  | T_t_s_10_1_s16.DataTypeOverride = 'Inherit';
  | T_t_s_10_1_s16.IsAlias = true;
  | 
  | T_t_s_10_1_u16 = Simulink.NumericType;
  | T_t_s_10_1_u16.Description = 's (seconds  (s))';
  | if (tmpVer > 7.11)
  | 	T_t_s_10_1_u16.DataScope = 'Auto';
  | end
  | T_t_s_10_1_u16.HeaderFile = 'Rte_Type.h';
  | T_t_s_10_1_u16.DataTypeMode = 'Fixed-point: slope and bias scaling';
  | T_t_s_10_1_u16.SignednessBool = false;
  | T_t_s_10_1_u16.WordLength = 16;
  | T_t_s_10_1_u16.FixedExponent = -4;
  | T_t_s_10_1_u16.SlopeAdjustmentFactor = 1.6;
  | T_t_s_10_1_u16.Bias = 0;
  | T_t_s_10_1_u16.DataTypeOverride = 'Inherit';
  | T_t_s_10_1_u16.IsAlias = true;
  | 
  | T_t_s_1_1_s16 = Simulink.NumericType;
  | T_t_s_1_1_s16.Description = 's (seconds  (s))';
  | if (tmpVer > 7.11)
  | 	T_t_s_1_1_s16.DataScope = 'Auto';
  | end
  | T_t_s_1_1_s16.HeaderFile = 'Rte_Type.h';
  | T_t_s_1_1_s16.DataTypeMode = 'Fixed-point: slope and bias scaling';
  | T_t_s_1_1_s16.SignednessBool = true;
  | T_t_s_1_1_s16.WordLength = 16;
  | T_t_s_1_1_s16.FixedExponent = 0;
  | T_t_s_1_1_s16.SlopeAdjustmentFactor = 1;
  | T_t_s_1_1_s16.Bias = 0;
  | T_t_s_1_1_s16.DataTypeOverride = 'Inherit';
  | T_t_s_1_1_s16.IsAlias = true;
  | 
  | T_t_s_1_1_u16 = Simulink.NumericType;
  | T_t_s_1_1_u16.Description = 's (seconds  (s))';
  | if (tmpVer > 7.11)
  | 	T_t_s_1_1_u16.DataScope = 'Auto';
  | end
  | T_t_s_1_1_u16.HeaderFile = 'Rte_Type.h';
  | T_t_s_1_1_u16.DataTypeMode = 'Fixed-point: slope and bias scaling';
  | T_t_s_1_1_u16.SignednessBool = false;
  | T_t_s_1_1_u16.WordLength = 16;
  | T_t_s_1_1_u16.FixedExponent = 0;
  | T_t_s_1_1_u16.SlopeAdjustmentFactor = 1;
  | T_t_s_1_1_u16.Bias = 0;
  | T_t_s_1_1_u16.DataTypeOverride = 'Inherit';
  | T_t_s_1_1_u16.IsAlias = true;
  | 
  | T_t_s_1_1_u32 = Simulink.NumericType;
  | T_t_s_1_1_u32.Description = 's (seconds  (s))';
  | if (tmpVer > 7.11)
  | 	T_t_s_1_1_u32.DataScope = 'Auto';
  | end
  | T_t_s_1_1_u32.HeaderFile = 'Rte_Type.h';
  | T_t_s_1_1_u32.DataTypeMode = 'Fixed-point: slope and bias scaling';
  | T_t_s_1_1_u32.SignednessBool = false;
  | T_t_s_1_1_u32.WordLength = 32;
  | T_t_s_1_1_u32.FixedExponent = 0;
  | T_t_s_1_1_u32.SlopeAdjustmentFactor = 1;
  | T_t_s_1_1_u32.Bias = 0;
  | T_t_s_1_1_u32.DataTypeOverride = 'Inherit';
  | T_t_s_1_1_u32.IsAlias = true;
  | 
  | T_t_s_Float32 = Simulink.NumericType;
  | T_t_s_Float32.Description = 's (seconds  (s))';
  | if (tmpVer > 7.11)
  | 	T_t_s_Float32.DataScope = 'Auto';
  | end
  | T_t_s_Float32.HeaderFile = 'Rte_Type.h';
  | T_t_s_Float32.DataTypeMode = 'Single';
  | T_t_s_Float32.SignednessBool = true;
  | T_t_s_Float32.WordLength = 32;
  | T_t_s_Float32.FixedExponent = 0;
  | T_t_s_Float32.SlopeAdjustmentFactor = 1;
  | T_t_s_Float32.Bias = 0;
  | T_t_s_Float32.DataTypeOverride = 'Inherit';
  | T_t_s_Float32.IsAlias = true;
  | 
  | T_t_us_10_1_u32 = Simulink.NumericType;
  | T_t_us_10_1_u32.Description = 'us (microseconds  (us))';
  | if (tmpVer > 7.11)
  | 	T_t_us_10_1_u32.DataScope = 'Auto';
  | end
  | T_t_us_10_1_u32.HeaderFile = 'Rte_Type.h';
  | T_t_us_10_1_u32.DataTypeMode = 'Fixed-point: slope and bias scaling';
  | T_t_us_10_1_u32.SignednessBool = false;
  | T_t_us_10_1_u32.WordLength = 32;
  | T_t_us_10_1_u32.FixedExponent = -4;
  | T_t_us_10_1_u32.SlopeAdjustmentFactor = 1.6;
  | T_t_us_10_1_u32.Bias = 0;
  | T_t_us_10_1_u32.DataTypeOverride = 'Inherit';
  | T_t_us_10_1_u32.IsAlias = true;
  | 
  | T_t_us_1_1_s16 = Simulink.NumericType;
  | T_t_us_1_1_s16.Description = 'us (microseconds  (us))';
  | if (tmpVer > 7.11)
  | 	T_t_us_1_1_s16.DataScope = 'Auto';
  | end
  | T_t_us_1_1_s16.HeaderFile = 'Rte_Type.h';
  | T_t_us_1_1_s16.DataTypeMode = 'Fixed-point: slope and bias scaling';
  | T_t_us_1_1_s16.SignednessBool = true;
  | T_t_us_1_1_s16.WordLength = 16;
  | T_t_us_1_1_s16.FixedExponent = 0;
  | T_t_us_1_1_s16.SlopeAdjustmentFactor = 1;
  | T_t_us_1_1_s16.Bias = 0;
  | T_t_us_1_1_s16.DataTypeOverride = 'Inherit';
  | T_t_us_1_1_s16.IsAlias = true;
  | 
  | T_t_us_1_1_u32 = Simulink.NumericType;
  | T_t_us_1_1_u32.Description = 'us (microseconds  (us))';
  | if (tmpVer > 7.11)
  | 	T_t_us_1_1_u32.DataScope = 'Auto';
  | end
  | T_t_us_1_1_u32.HeaderFile = 'Rte_Type.h';
  | T_t_us_1_1_u32.DataTypeMode = 'Fixed-point: slope and bias scaling';
  | T_t_us_1_1_u32.SignednessBool = false;
  | T_t_us_1_1_u32.WordLength = 32;
  | T_t_us_1_1_u32.FixedExponent = 0;
  | T_t_us_1_1_u32.SlopeAdjustmentFactor = 1;
  | T_t_us_1_1_u32.Bias = 0;
  | T_t_us_1_1_u32.DataTypeOverride = 'Inherit';
  | T_t_us_1_1_u32.IsAlias = true;
  | 
  | T_t_us_1_4_u16 = Simulink.NumericType;
  | T_t_us_1_4_u16.Description = 'us (microseconds  (us))';
  | if (tmpVer > 7.11)
  | 	T_t_us_1_4_u16.DataScope = 'Auto';
  | end
  | T_t_us_1_4_u16.HeaderFile = 'Rte_Type.h';
  | T_t_us_1_4_u16.DataTypeMode = 'Fixed-point: slope and bias scaling';
  | T_t_us_1_4_u16.SignednessBool = false;
  | T_t_us_1_4_u16.WordLength = 16;
  | T_t_us_1_4_u16.FixedExponent = 2;
  | T_t_us_1_4_u16.SlopeAdjustmentFactor = 1;
  | T_t_us_1_4_u16.Bias = 0;
  | T_t_us_1_4_u16.DataTypeOverride = 'Inherit';
  | T_t_us_1_4_u16.IsAlias = true;
  | 
  | T_t_us_Float32 = Simulink.NumericType;
  | T_t_us_Float32.Description = 'us (microseconds  (us))';
  | if (tmpVer > 7.11)
  | 	T_t_us_Float32.DataScope = 'Auto';
  | end
  | T_t_us_Float32.HeaderFile = 'Rte_Type.h';
  | T_t_us_Float32.DataTypeMode = 'Single';
  | T_t_us_Float32.SignednessBool = true;
  | T_t_us_Float32.WordLength = 32;
  | T_t_us_Float32.FixedExponent = 0;
  | T_t_us_Float32.SlopeAdjustmentFactor = 1;
  | T_t_us_Float32.Bias = 0;
  | T_t_us_Float32.DataTypeOverride = 'Inherit';
  | T_t_us_Float32.IsAlias = true;
  | 
  | T_v_kph_1_1_u8 = Simulink.NumericType;
  | T_v_kph_1_1_u8.Description = 'kph (kilometers / hour  (kph))';
  | if (tmpVer > 7.11)
  | 	T_v_kph_1_1_u8.DataScope = 'Auto';
  | end
  | T_v_kph_1_1_u8.HeaderFile = 'Rte_Type.h';
  | T_v_kph_1_1_u8.DataTypeMode = 'Fixed-point: slope and bias scaling';
  | T_v_kph_1_1_u8.SignednessBool = false;
  | T_v_kph_1_1_u8.WordLength = 8;
  | T_v_kph_1_1_u8.FixedExponent = 0;
  | T_v_kph_1_1_u8.SlopeAdjustmentFactor = 1;
  | T_v_kph_1_1_u8.Bias = 0;
  | T_v_kph_1_1_u8.DataTypeOverride = 'Inherit';
  | T_v_kph_1_1_u8.IsAlias = true;
  | 
  | T_v_kph_64_1_s16 = Simulink.NumericType;
  | T_v_kph_64_1_s16.Description = 'kph (kilometers / hour  (kph))';
  | if (tmpVer > 7.11)
  | 	T_v_kph_64_1_s16.DataScope = 'Auto';
  | end
  | T_v_kph_64_1_s16.HeaderFile = 'Rte_Type.h';
  | T_v_kph_64_1_s16.DataTypeMode = 'Fixed-point: slope and bias scaling';
  | T_v_kph_64_1_s16.SignednessBool = true;
  | T_v_kph_64_1_s16.WordLength = 16;
  | T_v_kph_64_1_s16.FixedExponent = -6;
  | T_v_kph_64_1_s16.SlopeAdjustmentFactor = 1;
  | T_v_kph_64_1_s16.Bias = 0;
  | T_v_kph_64_1_s16.DataTypeOverride = 'Inherit';
  | T_v_kph_64_1_s16.IsAlias = true;
  | 
  | T_v_kph_64_1_u16 = Simulink.NumericType;
  | T_v_kph_64_1_u16.Description = 'kph (kilometers / hour  (kph))';
  | if (tmpVer > 7.11)
  | 	T_v_kph_64_1_u16.DataScope = 'Auto';
  | end
  | T_v_kph_64_1_u16.HeaderFile = 'Rte_Type.h';
  | T_v_kph_64_1_u16.DataTypeMode = 'Fixed-point: slope and bias scaling';
  | T_v_kph_64_1_u16.SignednessBool = false;
  | T_v_kph_64_1_u16.WordLength = 16;
  | T_v_kph_64_1_u16.FixedExponent = -6;
  | T_v_kph_64_1_u16.SlopeAdjustmentFactor = 1;
  | T_v_kph_64_1_u16.Bias = 0;
  | T_v_kph_64_1_u16.DataTypeOverride = 'Inherit';
  | T_v_kph_64_1_u16.IsAlias = true;
  | 
  | T_v_kph_Float32 = Simulink.NumericType;
  | T_v_kph_Float32.Description = 'kph (kilometers / hour  (kph))';
  | if (tmpVer > 7.11)
  | 	T_v_kph_Float32.DataScope = 'Auto';
  | end
  | T_v_kph_Float32.HeaderFile = 'Rte_Type.h';
  | T_v_kph_Float32.DataTypeMode = 'Single';
  | T_v_kph_Float32.SignednessBool = true;
  | T_v_kph_Float32.WordLength = 32;
  | T_v_kph_Float32.FixedExponent = 0;
  | T_v_kph_Float32.SlopeAdjustmentFactor = 1;
  | T_v_kph_Float32.Bias = 0;
  | T_v_kph_Float32.DataTypeOverride = 'Inherit';
  | T_v_kph_Float32.IsAlias = true;
  | 
  | T_v_mps_256_1_s16 = Simulink.NumericType;
  | T_v_mps_256_1_s16.Description = 'mps (meters / second  (m/s))';
  | if (tmpVer > 7.11)
  | 	T_v_mps_256_1_s16.DataScope = 'Auto';
  | end
  | T_v_mps_256_1_s16.HeaderFile = 'Rte_Type.h';
  | T_v_mps_256_1_s16.DataTypeMode = 'Fixed-point: slope and bias scaling';
  | T_v_mps_256_1_s16.SignednessBool = true;
  | T_v_mps_256_1_s16.WordLength = 16;
  | T_v_mps_256_1_s16.FixedExponent = -8;
  | T_v_mps_256_1_s16.SlopeAdjustmentFactor = 1;
  | T_v_mps_256_1_s16.Bias = 0;
  | T_v_mps_256_1_s16.DataTypeOverride = 'Inherit';
  | T_v_mps_256_1_s16.IsAlias = true;
  | 
  | T_v_mps_Float32 = Simulink.NumericType;
  | T_v_mps_Float32.Description = 'mps (meters / second  (m/s))';
  | if (tmpVer > 7.11)
  | 	T_v_mps_Float32.DataScope = 'Auto';
  | end
  | T_v_mps_Float32.HeaderFile = 'Rte_Type.h';
  | T_v_mps_Float32.DataTypeMode = 'Single';
  | T_v_mps_Float32.SignednessBool = true;
  | T_v_mps_Float32.WordLength = 32;
  | T_v_mps_Float32.FixedExponent = 0;
  | T_v_mps_Float32.SlopeAdjustmentFactor = 1;
  | T_v_mps_Float32.Bias = 0;
  | T_v_mps_Float32.DataTypeOverride = 'Inherit';
  | T_v_mps_Float32.IsAlias = true;
  | 
  | T_w_radps_32_1_s16 = Simulink.NumericType;
  | T_w_radps_32_1_s16.Description = 'radps (radians / second  (rad/s))';
  | if (tmpVer > 7.11)
  | 	T_w_radps_32_1_s16.DataScope = 'Auto';
  | end
  | T_w_radps_32_1_s16.HeaderFile = 'Rte_Type.h';
  | T_w_radps_32_1_s16.DataTypeMode = 'Fixed-point: slope and bias scaling';
  | T_w_radps_32_1_s16.SignednessBool = true;
  | T_w_radps_32_1_s16.WordLength = 16;
  | T_w_radps_32_1_s16.FixedExponent = -5;
  | T_w_radps_32_1_s16.SlopeAdjustmentFactor = 1;
  | T_w_radps_32_1_s16.Bias = 0;
  | T_w_radps_32_1_s16.DataTypeOverride = 'Inherit';
  | T_w_radps_32_1_s16.IsAlias = true;
  | 
  | T_w_radps_Float32 = Simulink.NumericType;
  | T_w_radps_Float32.Description = 'radps (radians / second  (rad/s))';
  | if (tmpVer > 7.11)
  | 	T_w_radps_Float32.DataScope = 'Auto';
  | end
  | T_w_radps_Float32.HeaderFile = 'Rte_Type.h';
  | T_w_radps_Float32.DataTypeMode = 'Single';
  | T_w_radps_Float32.SignednessBool = true;
  | T_w_radps_Float32.WordLength = 32;
  | T_w_radps_Float32.FixedExponent = 0;
  | T_w_radps_Float32.SlopeAdjustmentFactor = 1;
  | T_w_radps_Float32.Bias = 0;
  | T_w_radps_Float32.DataTypeOverride = 'Inherit';
  | T_w_radps_Float32.IsAlias = true;
  | 
  | T_y_BitField8 = Simulink.NumericType;
  | T_y_BitField8.Description = 'BitField';
  | if (tmpVer > 7.11)
  | 	T_y_BitField8.DataScope = 'Auto';
  | end
  | T_y_BitField8.HeaderFile = 'Rte_Type.h';
  | T_y_BitField8.DataTypeMode = 'Fixed-point: slope and bias scaling';
  | T_y_BitField8.SignednessBool = false;
  | T_y_BitField8.WordLength = 8;
  | T_y_BitField8.FixedExponent = 0;
  | T_y_BitField8.SlopeAdjustmentFactor = 1;
  | T_y_BitField8.Bias = 0;
  | T_y_BitField8.DataTypeOverride = 'Inherit';
  | T_y_BitField8.IsAlias = true;
  | 
  | T_y_BitFieldDiagProgress = Simulink.NumericType;
  | T_y_BitFieldDiagProgress.Description = 'BitField';
  | if (tmpVer > 7.11)
  | 	T_y_BitFieldDiagProgress.DataScope = 'Auto';
  | end
  | T_y_BitFieldDiagProgress.HeaderFile = 'Rte_Type.h';
  | T_y_BitFieldDiagProgress.DataTypeMode = ...
  |   'Fixed-point: slope and bias scaling';
  | T_y_BitFieldDiagProgress.SignednessBool = false;
  | T_y_BitFieldDiagProgress.WordLength = 8;
  | T_y_BitFieldDiagProgress.FixedExponent = 0;
  | T_y_BitFieldDiagProgress.SlopeAdjustmentFactor = 1;
  | T_y_BitFieldDiagProgress.Bias = 0;
  | T_y_BitFieldDiagProgress.DataTypeOverride = 'Inherit';
  | T_y_BitFieldDiagProgress.IsAlias = true;
  | 
  | T_y_BitFieldDiagStatus = Simulink.NumericType;
  | T_y_BitFieldDiagStatus.Description = 'BitField';
  | if (tmpVer > 7.11)
  | 	T_y_BitFieldDiagStatus.DataScope = 'Auto';
  | end
  | T_y_BitFieldDiagStatus.HeaderFile = 'Rte_Type.h';
  | T_y_BitFieldDiagStatus.DataTypeMode = ...
  |   'Fixed-point: slope and bias scaling';
  | T_y_BitFieldDiagStatus.SignednessBool = false;
  | T_y_BitFieldDiagStatus.WordLength = 8;
  | T_y_BitFieldDiagStatus.FixedExponent = 0;
  | T_y_BitFieldDiagStatus.SlopeAdjustmentFactor = 1;
  | T_y_BitFieldDiagStatus.Bias = 0;
  | T_y_BitFieldDiagStatus.DataTypeOverride = 'Inherit';
  | T_y_BitFieldDiagStatus.IsAlias = true;
  | 
  | T_y_NA_1_1_u8 = Simulink.NumericType;
  | T_y_NA_1_1_u8.Description = 'TYPE TO BE REMOVED';
  | if (tmpVer > 7.11)
  | 	T_y_NA_1_1_u8.DataScope = 'Auto';
  | end
  | T_y_NA_1_1_u8.HeaderFile = 'Rte_Type.h';
  | T_y_NA_1_1_u8.DataTypeMode = 'Fixed-point: slope and bias scaling';
  | T_y_NA_1_1_u8.SignednessBool = false;
  | T_y_NA_1_1_u8.WordLength = 8;
  | T_y_NA_1_1_u8.FixedExponent = 0;
  | T_y_NA_1_1_u8.SlopeAdjustmentFactor = 1;
  | T_y_NA_1_1_u8.Bias = 0;
  | T_y_NA_1_1_u8.DataTypeOverride = 'Inherit';
  | T_y_NA_1_1_u8.IsAlias = true;
  | 
  | UInt16 = Simulink.AliasType;
  | UInt16.Description = 'Num';
  | if (tmpVer > 7.11)
  | 	UInt16.DataScope = 'Auto';
  | end
  | UInt16.HeaderFile = 'Rte_Type.h';
  | UInt16.BaseType = 'uint16';
  | 
  | UInt32 = Simulink.AliasType;
  | UInt32.Description = 'Num';
  | if (tmpVer > 7.11)
  | 	UInt32.DataScope = 'Auto';
  | end
  | UInt32.HeaderFile = 'Rte_Type.h';
  | UInt32.BaseType = 'uint32';
  | 
  | UInt8 = Simulink.AliasType;
  | UInt8.Description = 'Num';
  | if (tmpVer > 7.11)
  | 	UInt8.DataScope = 'Auto';
  | end
  | UInt8.HeaderFile = 'Rte_Type.h';
  | UInt8.BaseType = 'uint8';
  | 
  | s16 = Simulink.AliasType;
  | s16.Description = 'TYPE TO BE REMOVED';
  | if (tmpVer > 7.11)
  | 	s16.DataScope = 'Auto';
  | end
  | s16.HeaderFile = 'Rte_Type.h';
  | s16.BaseType = 'int16';
  | 
  | s32 = Simulink.AliasType;
  | s32.Description = 'TYPE TO BE REMOVED';
  | if (tmpVer > 7.11)
  | 	s32.DataScope = 'Auto';
  | end
  | s32.HeaderFile = 'Rte_Type.h';
  | s32.BaseType = 'int32';
  | 
  | s8 = Simulink.AliasType;
  | s8.Description = 'TYPE TO BE REMOVED';
  | if (tmpVer > 7.11)
  | 	s8.DataScope = 'Auto';
  | end
  | s8.HeaderFile = 'Rte_Type.h';
  | s8.BaseType = 'int8';
  | 
  | u16 = Simulink.AliasType;
  | u16.Description = 'TYPE TO BE REMOVED';
  | if (tmpVer > 7.11)
  | 	u16.DataScope = 'Auto';
  | end
  | u16.HeaderFile = 'Rte_Type.h';
  | u16.BaseType = 'uint16';
  | 
  | u32 = Simulink.AliasType;
  | u32.Description = 'TYPE TO BE REMOVED';
  | if (tmpVer > 7.11)
  | 	u32.DataScope = 'Auto';
  | end
  | u32.HeaderFile = 'Rte_Type.h';
  | u32.BaseType = 'uint32';
  | 
  | u8 = Simulink.AliasType;
  | u8.Description = 'TYPE TO BE REMOVED';
  | if (tmpVer > 7.11)
  | 	u8.DataScope = 'Auto';
  | end
  | u8.HeaderFile = 'Rte_Type.h';
  | u8.BaseType = 'uint8';
  | 
  | clear tmpVer
  | 
  | 
  | ob_LKA_Disable_Reason = Simulink.Signal;
  | ob_LKA_Disable_Reason.CoderInfo.StorageClass = 'Custom';
  | ob_LKA_Disable_Reason.CoderInfo.Alias = '';
  | ob_LKA_Disable_Reason.CoderInfo.Alignment = -1;
  | ob_LKA_Disable_Reason.CoderInfo.CustomStorageClass = 'Default';
  | ob_LKA_Disable_Reason.Description = '';
  | ob_LKA_Disable_Reason.DataType = 'single';
  | ob_LKA_Disable_Reason.Min = [];
  | ob_LKA_Disable_Reason.Max = [];
  | ob_LKA_Disable_Reason.DocUnits = '';
  | ob_LKA_Disable_Reason.Dimensions = -1;
  | ob_LKA_Disable_Reason.DimensionsMode = 'auto';
  | ob_LKA_Disable_Reason.Complexity = 'auto';
  | ob_LKA_Disable_Reason.SampleTime = -1;
  | ob_LKA_Disable_Reason.InitialValue = '';
  | 
  | ob_LKA_LKADeactvCSyn = Simulink.Signal;
  | ob_LKA_LKADeactvCSyn.CoderInfo.StorageClass = 'Custom';
  | ob_LKA_LKADeactvCSyn.CoderInfo.Alias = '';
  | ob_LKA_LKADeactvCSyn.CoderInfo.Alignment = -1;
  | ob_LKA_LKADeactvCSyn.CoderInfo.CustomStorageClass = 'Default';
  | ob_LKA_LKADeactvCSyn.Description = '';
  | ob_LKA_LKADeactvCSyn.DataType = 'single';
  | ob_LKA_LKADeactvCSyn.Min = [];
  | ob_LKA_LKADeactvCSyn.Max = [];
  | ob_LKA_LKADeactvCSyn.DocUnits = '';
  | ob_LKA_LKADeactvCSyn.Dimensions = -1;
  | ob_LKA_LKADeactvCSyn.DimensionsMode = 'auto';
  | ob_LKA_LKADeactvCSyn.Complexity = 'auto';
  | ob_LKA_LKADeactvCSyn.SampleTime = -1;
  | ob_LKA_LKADeactvCSyn.InitialValue = '';
  | 
  | ob_LKA_Version = Simulink.Signal;
  | ob_LKA_Version.CoderInfo.StorageClass = 'Custom';
  | ob_LKA_Version.CoderInfo.Alias = '';
  | ob_LKA_Version.CoderInfo.Alignment = -1;
  | ob_LKA_Version.CoderInfo.CustomStorageClass = 'Default';
  | ob_LKA_Version.Description = '';
  | ob_LKA_Version.DataType = 'single';
  | ob_LKA_Version.Min = [];
  | ob_LKA_Version.Max = [];
  | ob_LKA_Version.DocUnits = '';
  | ob_LKA_Version.Dimensions = -1;
  | ob_LKA_Version.DimensionsMode = 'auto';
  | ob_LKA_Version.Complexity = 'auto';
  | ob_LKA_Version.SampleTime = -1;
  | ob_LKA_Version.InitialValue = '';
StopFcn:
  | clear  T_A_m2_1024_1_u32 T_A_m2_65536_1_u16 T_A_m2_Float32 T_A_mm2_10_1_u16 T_A_mm2_4_1_s16 T_A_mm2_Float32 T_Cnt_Num_10_1_u32 T_Cnt_Num_1_1_s16 T_Cnt_Num_1_1_s32 T_Cnt_Num_1_1_s8 T_Cnt_Num_1_1_u16 T_Cnt_Num_1_1_u32 T_Cnt_Num_1_1_u8 T_E_J_1_1_s32 T_E_J_Float32 T_E_kJ_128_1_s32 T_E_kJ_Float32 T_E_kwh_10_1_u16 T_E_kwh_Float32 T_Epl_kwhpkm_100_1_u16 T_Epl_kwhpkm_Float32 T_F_N_1_1_s16 T_F_N_Float32 T_I_A_1000_1_u16 T_I_A_1048576_1_s32 T_I_A_2048_1_s16 T_I_A_32_1_s16 T_I_A_Float32 T_I_mA_1_1_s16 T_I_mA_32768_128_s16 T_I_mA_Float32 T_J_kgpm2_128_1_u16 T_J_kgpm2_Float32 T_K_NA_1000_1_s16 T_K_NA_100_1_s16 T_K_NA_100_1_u16 T_K_NA_1024_1_s16 T_K_NA_1024_1_u16 T_K_NA_128_1_s16 T_K_NA_128_1_u16 T_K_NA_128_1_u8 T_K_NA_16777216_1_u32 T_K_NA_16_1_s16 T_K_NA_16_1_u16 T_K_NA_16_1_u8 T_K_NA_1_16_u16 T_K_NA_1_1_s16 T_K_NA_1_1_u16 T_K_NA_1_1_u8 T_K_NA_32768_1_s16 T_K_NA_32768_1_u16 T_K_NA_32_1_s8 T_K_NA_4096_1_u16 T_K_NA_4194304_1_s32 T_K_NA_4194304_1_u16 T_K_NA_65536_1_s32 T_K_NA_65536_1_u16 T_K_NA_8192_1_s16 T_K_NA_8_1_s16 T_K_NA_Float32 T_M_Nm_16_1_s16 T_M_Nm_1_1_s16 T_M_Nm_32768_1_s16 T_M_Nm_32_1_s16 T_M_Nm_4_1_s16 T_M_Nm_512_1_s16 T_M_Nm_Float32 T_P_W_1_4_s16 T_P_W_1_8_s16 T_P_W_Float32 T_P_kW_128_1_s16 T_P_kW_1_8_s16 T_P_kW_8_1_s32 T_P_kW_Float32 T_Pct_pct_1024_1_s32 T_Pct_pct_1024_1_u32 T_Pct_pct_10_1_s16 T_Pct_pct_10_1_u32 T_Pct_pct_128_100_s8 T_Pct_pct_1_1_s16 T_Pct_pct_1_4_u8 T_Pct_pct_255_100_u16 T_Pct_pct_255_100_u8 T_Pct_pct_256_1_s16 T_Pct_pct_256_1_u16 T_Pct_pct_65535_100_u16 T_Pct_pct_Float32 T_R_ohm_1024_1_s16 T_R_ohm_32_1_s16 T_R_ohm_Float32 T_TK_K_16_1_s16 T_TK_K_Float32 T_T_degC_10_400_1_u16 T_T_degC_16_1_s16 T_T_degC_1_40_1_u8 T_T_degC_2_80_1_u8 T_T_degC_Float32 T_U_V_1000_1_u16 T_U_V_10_1_u8 T_U_V_200_1_u8 T_U_V_32_1_s16 T_U_V_4096_1_s16 T_U_V_512_1_s16 T_U_V_65535_8_u16 T_U_V_8192_1_u16 T_U_V_Float32 T_U_mV_1_1_s16 T_U_mV_256_20_u16 T_U_mV_Float32 T_V_l_256_1_s16 T_V_l_4096_1_s16 T_V_l_64_1_s16 T_V_l_65535_100_u16 T_V_l_Float32 T_V_ml_128_1_s16 T_V_ml_1_1_s16 T_V_ml_32768_1_s16 T_V_ml_Float32 T_V_ul_32_1_u16 T_V_ul_Float32 T_Vpl_clpkm_512_1_u16 T_Vpl_clpkm_Float32 T_a_kphps_16_1_s16 T_a_kphps_Float32 T_a_mps2_128_1_s16 T_a_mps2_Float32 T_c_MJpkg_256_1_s16 T_c_MJpkg_Float32 T_c_kJpgpK_1024_1_s16 T_c_kJpgpK_Float32 T_c_kJpkgpK_128_1_u16 T_c_kJpkgpK_Float32 T_chrg_Ah_1_1_s16 T_chrg_Ah_1_1_u16 T_chrg_Ah_1_1_u8 T_chrg_Ah_256_1_u16 T_chrg_Ah_4194304_1_s32 T_chrg_Ah_512_1_u16 T_chrg_Ah_8_1_u16 T_chrg_Ah_Float32 T_cmp_NA_100_1_s16 T_cmp_NA_128_1_s16 T_cmp_NA_16_1_s16 T_cmp_NA_32768_1_u16 T_cmp_NA_Float32 T_d2n_rpmps2_4_1_s16 T_d2n_rpmps2_Float32 T_dPct_pctps_16_1_s16 T_dPct_pctps_256_1_s16 T_dPct_pctps_Float32 T_dT_degCps_128_1_s16 T_dT_degCps_Float32 T_dV_lph_1_1_s16 T_dV_lph_Float32 T_dV_lpm_128_1_s16 T_dV_lpm_32_1_s16 T_dV_lpm_Float32 T_dV_lps_1024_1_u16 T_dV_lps_4_1_u16 T_dV_lps_Float32 T_dV_mlps_1024_1_s16 T_dV_mlps_Float32 T_d_BitField16 T_dm_gps_128_1_s16 T_dm_gps_128_1_u16 T_dm_gps_256_1_u16 T_dm_gps_Float32 T_dm_mgps_1_1_s16 T_dm_mgps_Float32 T_dn_rpmps_1_1_s16 T_dn_rpmps_2_1_s16 T_dn_rpmps_Float32 T_dp_Paps_1_1_s16 T_dp_Paps_Float32 T_dp_kPaps_1_1_s16 T_dp_kPaps_8_1_s16 T_dp_kPaps_Float32 T_dphi_degps_128_1_s16 T_dphi_degps_8_1_s16 T_dphi_degps_Float32 T_dr_ps_256_1_s16 T_dr_ps_Float32 T_drho_mgplps_1_2_s16 T_drho_mgplps_Float32 T_e_NA_1_1_u8 T_f_Hz_1_1_u16 T_f_Hz_1_1_u32 T_f_Hz_64_1_u16 T_f_Hz_8_1_s16 T_f_Hz_Float32 T_g_BitField32 T_l_km_16_1_s16 T_l_km_1_1_u16 T_l_km_1_1_u32 T_l_km_Float32 T_l_m_1024_1_s16 T_l_m_16_1_s16 T_l_m_1_1_u32 T_l_m_Float32 T_l_mm_16_1_s16 T_l_mm_1_1_u16 T_l_mm_4096_1_s16 T_l_mm_4_1_u8 T_l_mm_64_1_s16 T_l_mm_Float32 T_m_g_1_1_s16 T_m_g_2048_1_s16 T_m_g_32_1_u16 T_m_g_Float32 T_m_kg_1024_1_s16 T_m_kg_1_1_s16 T_m_kg_1_1_u32 T_m_kg_Float32 T_m_mg_128_1_s16 T_m_mg_32_1_s16 T_m_mg_Float32 T_n_rpm_1_1_s16 T_n_rpm_1_25_u8 T_n_rpm_256_50_u16 T_n_rpm_2_25_u8 T_n_rpm_4_1_u16 T_n_rpm_Float32 T_p_MPa_64_1_s16 T_p_MPa_Float32 T_p_Pa_1_1_s16 T_p_Pa_Float32 T_p_kPa_1_10_u16 T_p_kPa_1_1_s16 T_p_kPa_1_1_u8 T_p_kPa_256_1_u16 T_p_kPa_32_1_u16 T_p_kPa_64_1_s16 T_p_kPa_Float32 T_phi_deg_100_1_s16 T_phi_deg_1024_1_s16 T_phi_deg_128_1_s16 T_phi_deg_1_1_u8 T_phi_deg_256_1_s16 T_phi_deg_2_1_s8 T_phi_deg_32_1_s16 T_phi_deg_512_6_s32 T_phi_deg_Float32 T_phi_rad_2048_1_s16 T_phi_rad_Float32 T_r_NA_1024_1_s16 T_r_NA_1024_1_u16 T_r_NA_16384_1_s16 T_r_NA_16_1_s16 T_r_NA_256_1_s8 T_r_NA_256_1_u16 T_r_NA_32768_1_u16 T_r_NA_32_1_u16 T_r_NA_4096_1_s16 T_r_NA_65535_2_u16 T_r_NA_8192_1_u16 T_r_NA_Float32 T_rho_gpl_8192_1_s16 T_rho_gpl_Float32 T_rho_kgpm3_16_1_s16 T_rho_kgpm3_Float32 T_rho_mgpl_1_1_s16 T_rho_mgpl_64_1_s16 T_rho_mgpl_Float32 T_t_hour_1_1_s16 T_t_hour_Float32 T_t_m_1_1_u16 T_t_m_Float32 T_t_ms_1_1_s16 T_t_ms_1_1_u16 T_t_ms_1_1_u32 T_t_ms_4096_1_s16 T_t_ms_64_1_s16 T_t_ms_Float32 T_t_s_1000_1_s16 T_t_s_100_1_s16 T_t_s_10_1_s16 T_t_s_10_1_u16 T_t_s_1_1_s16 T_t_s_1_1_u16 T_t_s_1_1_u32 T_t_s_Float32 T_t_us_10_1_u32 T_t_us_1_1_s16 T_t_us_1_1_u32 T_t_us_1_4_u16 T_t_us_Float32 T_v_kph_1_1_u8 T_v_kph_64_1_s16 T_v_kph_64_1_u16 T_v_kph_Float32 T_v_mps_256_1_s16 T_v_mps_Float32 T_w_radps_32_1_s16 T_w_radps_Float32 T_y_BitField8 T_y_BitFieldDiagProgress T_y_BitFieldDiagStatus T_y_NA_1_1_u8 SInt16 SInt32 SInt8 T_BOOLEAN UInt16 UInt32 UInt8 s16 s32 s8 u16 u32 u8
model workspace (MAT data in the model file):
  LKA_CarWidth = Simulink.Parameter
  LKA_CarWidth.Value = 1.88
  LKA_CarWidth.DataType = 'single'
  LKA_CarWidth.Dimensions = [1 1]
  LKA_SampleTime = Simulink.Parameter
  LKA_SampleTime.Value = 0.01
  LKA_SampleTime.DataType = 'single'
  LKA_SampleTime.Dimensions = [1 1]
  LKA_StrRatio_C = Simulink.Parameter
  LKA_StrRatio_C.Value = 14.3
  LKA_StrRatio_C.DataType = 'single'
  LKA_StrRatio_C.Dimensions = [1 1]
  LKA_Veh2CamL_C = Simulink.Parameter
  LKA_Veh2CamL_C.Value = 1.73
  LKA_Veh2CamL_C.DataType = 'single'
  LKA_Veh2CamL_C.Dimensions = [1 1]
  LKA_Veh2CamW_C = Simulink.Parameter
  LKA_Veh2CamW_C.Value = 0.94
  LKA_Veh2CamW_C.DataType = 'single'
  LKA_Veh2CamW_C.Dimensions = [1 1]
  LKA_WhlBaseL_C = Simulink.Parameter
  LKA_WhlBaseL_C.Value = 2.8
  LKA_WhlBaseL_C.DataType = 'single'
  LKA_WhlBaseL_C.Dimensions = [1 1]
  LL_CompHdAg_C = Simulink.Parameter
  LL_CompHdAg_C.Value = 0
  LL_CompHdAg_C.DataType = 'single'
  LL_CompHdAg_C.Dimensions = [1 1]
  LL_CompSWA_C = Simulink.Parameter
  LL_CompSWA_C.Value = 0
  LL_CompSWA_C.DataType = 'single'
  LL_CompSWA_C.Dimensions = [1 1]
  LL_CrvtPrvwT_C = Simulink.Parameter
  LL_CrvtPrvwT_C.Value = 0.45
  LL_CrvtPrvwT_C.DataType = 'single'
  LL_CrvtPrvwT_C.Dimensions = [1 1]
  LL_DesDvt_C = Simulink.Parameter
  LL_DesDvt_C.Value = 0.2
  LL_DesDvt_C.DataType = 'single'
  LL_DesDvt_C.Dimensions = [1 1]
  LL_DvtComp_C = Simulink.Parameter
  LL_DvtComp_C.Value = 0
  LL_DvtComp_C.DataType = 'single'
  LL_DvtComp_C.Dimensions = [1 1]
  LL_DvtPrvwT_C = Simulink.Parameter
  LL_DvtPrvwT_C.Value = 0.45
  LL_DvtPrvwT_C.DataType = 'single'
  LL_DvtPrvwT_C.Dimensions = [1 1]
  LL_DvtSpdDet_vDvtSpdMin_C = Simulink.Parameter
  LL_DvtSpdDet_vDvtSpdMin_C.Value = 0
  LL_DvtSpdDet_vDvtSpdMin_C.DataType = 'single'
  LL_DvtSpdDet_vDvtSpdMin_C.Dimensions = [1 1]
  LL_HandsOff_ExitTime = Simulink.Parameter
  LL_HandsOff_ExitTime.Value = 10
  LL_HandsOff_ExitTime.DataType = 'single'
  LL_HandsOff_ExitTime.Dimensions = [1 1]
  LL_HandsOff_TextTime = Simulink.Parameter
  LL_HandsOff_TextTime.Value = 5
  LL_HandsOff_TextTime.DataType = 'single'
  LL_HandsOff_TextTime.Dimensions = [1 1]
  LL_HandsOff_WarnTime = Simulink.Parameter
  LL_HandsOff_WarnTime.Value = 5
  LL_HandsOff_WarnTime.DataType = 'single'
  LL_HandsOff_WarnTime.Dimensions = [1 1]
  LL_HdAgExT_C = Simulink.Parameter
  LL_HdAgExT_C.Value = 15
  LL_HdAgExT_C.DataType = 'single'
  LL_HdAgExT_C.Dimensions = [1 1]
  LL_HdAgPrvwT_C = Simulink.Parameter
  LL_HdAgPrvwT_C.Value = 0.45
  LL_HdAgPrvwT_C.DataType = 'single'
  LL_HdAgPrvwT_C.Dimensions = [1 1]
  LL_LAccMax_C = Simulink.Parameter
  LL_LAccMax_C.Value = 3
  LL_LAccMax_C.DataType = 'single'
  LL_LAccMax_C.Dimensions = [1 1]
  LL_LAccRMax_C = Simulink.Parameter
  LL_LAccRMax_C.Value = 5
  LL_LAccRMax_C.DataType = 'single'
  LL_LAccRMax_C.Dimensions = [1 1]
  LL_LDWS_SUPPRESS_HEADING = Simulink.Parameter
  LL_LDWS_SUPPRESS_HEADING.Value = 2
  LL_LDWS_SUPPRESS_HEADING.DataType = 'single'
  LL_LDWS_SUPPRESS_HEADING.Dimensions = [1 1]
  LL_LDW_EarliestWarnLine_C = Simulink.Parameter
  LL_LDW_EarliestWarnLine_C.Value = 0.3
  LL_LDW_EarliestWarnLine_C.DataType = 'single'
  LL_LDW_EarliestWarnLine_C.Dimensions = [1 1]
  LL_LDW_LatestWarnLine_C = Simulink.Parameter
  LL_LDW_LatestWarnLine_C.Value = -0.4
  LL_LDW_LatestWarnLine_C.DataType = 'single'
  LL_LDW_LatestWarnLine_C.Dimensions = [1 1]
  LL_LFClb_TFC_FfCtlRatio_C = Simulink.Parameter
  LL_LFClb_TFC_FfCtlRatio_C.Value = 1
  LL_LFClb_TFC_FfCtlRatio_C.DataType = 'single'
  LL_LFClb_TFC_FfCtlRatio_C.Dimensions = [1 1]
  LL_LFClb_TFC_KdBalance_C = Simulink.Parameter
  LL_LFClb_TFC_KdBalance_C.Value = 0
  LL_LFClb_TFC_KdBalance_C.DataType = 'single'
  LL_LFClb_TFC_KdBalance_C.Dimensions = [1 1]
  LL_LFClb_TFC_KdMaxSWA_C = Simulink.Parameter
  LL_LFClb_TFC_KdMaxSWA_C.Value = 20
  LL_LFClb_TFC_KdMaxSWA_C.DataType = 'single'
  LL_LFClb_TFC_KdMaxSWA_C.Dimensions = [1 1]
  LL_LFClb_TFC_KdV1_C = Simulink.Parameter
  LL_LFClb_TFC_KdV1_C.Value = 250
  LL_LFClb_TFC_KdV1_C.DataType = 'single'
  LL_LFClb_TFC_KdV1_C.Dimensions = [1 1]
  LL_LFClb_TFC_KdV2_C = Simulink.Parameter
  LL_LFClb_TFC_KdV2_C.Value = 250
  LL_LFClb_TFC_KdV2_C.DataType = 'single'
  LL_LFClb_TFC_KdV2_C.Dimensions = [1 1]
  LL_LFClb_TFC_KdVehSpdLwr_C = Simulink.Parameter
  LL_LFClb_TFC_KdVehSpdLwr_C.Value = 60
  LL_LFClb_TFC_KdVehSpdLwr_C.DataType = 'single'
  LL_LFClb_TFC_KdVehSpdLwr_C.Dimensions = [1 1]
  LL_LFClb_TFC_KdVehSpdUpr_C = Simulink.Parameter
  LL_LFClb_TFC_KdVehSpdUpr_C.Value = 120
  LL_LFClb_TFC_KdVehSpdUpr_C.DataType = 'single'
  LL_LFClb_TFC_KdVehSpdUpr_C.Dimensions = [1 1]
  LL_LFClb_TFC_KiMaxSWA_C = Simulink.Parameter
  LL_LFClb_TFC_KiMaxSWA_C.Value = 5
  LL_LFClb_TFC_KiMaxSWA_C.DataType = 'single'
  LL_LFClb_TFC_KiMaxSWA_C.Dimensions = [1 1]
  LL_LFClb_TFC_Ki_C = Simulink.Parameter
  LL_LFClb_TFC_Ki_C.Value = 0.002
  LL_LFClb_TFC_Ki_C.DataType = 'single'
  LL_LFClb_TFC_Ki_C.Dimensions = [1 1]
  LL_LFClb_TFC_KpKlat_C = Simulink.Parameter
  LL_LFClb_TFC_KpKlat_C.Value = -4.5
  LL_LFClb_TFC_KpKlat_C.DataType = 'single'
  LL_LFClb_TFC_KpKlat_C.Dimensions = [1 1]
  LL_LFClb_TFC_KpV1_C = Simulink.Parameter
  LL_LFClb_TFC_KpV1_C.Value = 40
  LL_LFClb_TFC_KpV1_C.DataType = 'single'
  LL_LFClb_TFC_KpV1_C.Dimensions = [1 1]
  LL_LFClb_TFC_KpV2_C = Simulink.Parameter
  LL_LFClb_TFC_KpV2_C.Value = 40
  LL_LFClb_TFC_KpV2_C.DataType = 'single'
  LL_LFClb_TFC_KpV2_C.Dimensions = [1 1]
  LL_LFClb_TFC_KpVehSpdLwr_C = Simulink.Parameter
  LL_LFClb_TFC_KpVehSpdLwr_C.Value = 60
  LL_LFClb_TFC_KpVehSpdLwr_C.DataType = 'single'
  LL_LFClb_TFC_KpVehSpdLwr_C.Dimensions = [1 1]
  LL_LFClb_TFC_KpVehSpdUpr_C = Simulink.Parameter
  LL_LFClb_TFC_KpVehSpdUpr_C.Value = 120
  LL_LFClb_TFC_KpVehSpdUpr_C.DataType = 'single'
  LL_LFClb_TFC_KpVehSpdUpr_C.Dimensions = [1 1]
  LL_LFClb_TFC_Kp_C = Simulink.Parameter
  LL_LFClb_TFC_Kp_C.Value = 1
  LL_LFClb_TFC_Kp_C.DataType = 'single'
  LL_LFClb_TFC_Kp_C.Dimensions = [1 1]
  LL_LFClb_TFC_PrvwT_C = Simulink.Parameter
  LL_LFClb_TFC_PrvwT_C.Value = 2
  LL_LFClb_TFC_PrvwT_C.DataType = 'single'
  LL_LFClb_TFC_PrvwT_C.Dimensions = [1 1]
  LL_LKAExPrcs_ExitC0Dvt = Simulink.Parameter
  LL_LKAExPrcs_ExitC0Dvt.Value = 0.06
  LL_LKAExPrcs_ExitC0Dvt.DataType = 'single'
  LL_LKAExPrcs_ExitC0Dvt.Dimensions = [1 1]
  LL_LKAExPrcs_ExitC0Swt = Simulink.Parameter
  LL_LKAExPrcs_ExitC0Swt.Value = 1
  LL_LKAExPrcs_ExitC0Swt.DataType = 'boolean'
  LL_LKAExPrcs_ExitC0Swt.Dimensions = [1 1]
  LL_LKAExPrcs_tiExitTime1 = Simulink.Parameter
  LL_LKAExPrcs_tiExitTime1.Value = 8
  LL_LKAExPrcs_tiExitTime1.DataType = 'single'
  LL_LKAExPrcs_tiExitTime1.Dimensions = [1 1]
  LL_LKAExPrcs_tiExitTime2 = Simulink.Parameter
  LL_LKAExPrcs_tiExitTime2.Value = 4
  LL_LKAExPrcs_tiExitTime2.DataType = 'single'
  LL_LKAExPrcs_tiExitTime2.Dimensions = [1 1]
  LL_LKAExPrcs_tiExitTime3 = Simulink.Parameter
  LL_LKAExPrcs_tiExitTime3.Value = 0.2
  LL_LKAExPrcs_tiExitTime3.DataType = 'single'
  LL_LKAExPrcs_tiExitTime3.Dimensions = [1 1]
  LL_LKASWASyn_M0 = Simulink.Parameter
  LL_LKASWASyn_M0.Value = 0.35
  LL_LKASWASyn_M0.DataType = 'single'
  LL_LKASWASyn_M0.Dimensions = [1 1]
  LL_LKASWASyn_M1 = Simulink.Parameter
  LL_LKASWASyn_M1.Value = 0.6
  LL_LKASWASyn_M1.DataType = 'single'
  LL_LKASWASyn_M1.Dimensions = [1 1]
  LL_LKASWASyn_M2 = Simulink.Parameter
  LL_LKASWASyn_M2.Value = 0.3
  LL_LKASWASyn_M2.DataType = 'single'
  LL_LKASWASyn_M2.Dimensions = [1 1]
  LL_LKASWASyn_M3K = Simulink.Parameter
  LL_LKASWASyn_M3K.Value = 0.2
  LL_LKASWASyn_M3K.DataType = 'single'
  LL_LKASWASyn_M3K.Dimensions = [1 1]
  LL_LKASWASyn_SWAaddMax = Simulink.Parameter
  LL_LKASWASyn_SWAaddMax.Value = 8
  LL_LKASWASyn_SWAaddMax.DataType = 'single'
  LL_LKASWASyn_SWAaddMax.Dimensions = [1 1]
  LL_LKASWASyn_T2 = Simulink.Parameter
  LL_LKASWASyn_T2.Value = 4
  LL_LKASWASyn_T2.DataType = 'single'
  LL_LKASWASyn_T2.Dimensions = [1 1]
  LL_LKASWASyn_TrqMax = Simulink.Parameter
  LL_LKASWASyn_TrqMax.Value = 1.5
  LL_LKASWASyn_TrqMax.DataType = 'single'
  LL_LKASWASyn_TrqMax.Dimensions = [1 1]
  LL_LKASWASyn_TrqSwaAddSwt = Simulink.Parameter
  LL_LKASWASyn_TrqSwaAddSwt.Value = 0
  LL_LKASWASyn_TrqSwaAddSwt.DataType = 'boolean'
  LL_LKASWASyn_TrqSwaAddSwt.Dimensions = [1 1]
  LL_LKASWASyn_TrqSwaRateDiff = Simulink.Parameter
  LL_LKASWASyn_TrqSwaRateDiff.Value = -0.2
  LL_LKASWASyn_TrqSwaRateDiff.DataType = 'single'
  LL_LKASWASyn_TrqSwaRateDiff.Dimensions = [1 1]
  LL_LKASWASyn_tiTrqSwaRtTime = Simulink.Parameter
  LL_LKASWASyn_tiTrqSwaRtTime.Value = 0.2
  LL_LKASWASyn_tiTrqSwaRtTime.DataType = 'single'
  LL_LKASWASyn_tiTrqSwaRtTime.Dimensions = [1 1]
  LL_LKASWASyn_tiTrqSwaTime = Simulink.Parameter
  LL_LKASWASyn_tiTrqSwaTime.Value = 0.3
  LL_LKASWASyn_tiTrqSwaTime.DataType = 'single'
  LL_LKASWASyn_tiTrqSwaTime.Dimensions = [1 1]
  LL_LKAS_OUT_OF_CONTROL_LAT_VEL = Simulink.Parameter
  LL_LKAS_OUT_OF_CONTROL_LAT_VEL.Value = 1.5
  LL_LKAS_OUT_OF_CONTROL_LAT_VEL.DataType = 'single'
  LL_LKAS_OUT_OF_CONTROL_LAT_VEL.Dimensions = [1 1]
  LL_LKAS_OUT_OF_CONTROL_TTLC = Simulink.Parameter
  LL_LKAS_OUT_OF_CONTROL_TTLC.Value = 0.3
  LL_LKAS_OUT_OF_CONTROL_TTLC.DataType = 'single'
  LL_LKAS_OUT_OF_CONTROL_TTLC.Dimensions = [1 1]
  LL_LKA_EarliestWarnLine_C = Simulink.Parameter
  LL_LKA_EarliestWarnLine_C.Value = 0.3
  LL_LKA_EarliestWarnLine_C.DataType = 'single'
  LL_LKA_EarliestWarnLine_C.Dimensions = [1 1]
  LL_LKA_LatestWarnLine_C = Simulink.Parameter
  LL_LKA_LatestWarnLine_C.Value = -0.5
  LL_LKA_LatestWarnLine_C.DataType = 'single'
  LL_LKA_LatestWarnLine_C.Dimensions = [1 1]
  LL_LSpdCompT_C = Simulink.Parameter
  LL_LSpdCompT_C.Value = 0.4
  LL_LSpdCompT_C.DataType = 'single'
  LL_LSpdCompT_C.Dimensions = [1 1]
  LL_MAX_DELAY_EPSSTAR_TIME = Simulink.Parameter
  LL_MAX_DELAY_EPSSTAR_TIME.Value = 0.5
  LL_MAX_DELAY_EPSSTAR_TIME.DataType = 'single'
  LL_MAX_DELAY_EPSSTAR_TIME.Dimensions = [1 1]
  LL_MAX_DRIVER_TORQUE_DISABLE = Simulink.Parameter
  LL_MAX_DRIVER_TORQUE_DISABLE.Value = 2.25
  LL_MAX_DRIVER_TORQUE_DISABLE.DataType = 'single'
  LL_MAX_DRIVER_TORQUE_DISABLE.Dimensions = [1 1]
  LL_MAX_DRIVER_TORQUE_ENABLE = Simulink.Parameter
  LL_MAX_DRIVER_TORQUE_ENABLE.Value = 3
  LL_MAX_DRIVER_TORQUE_ENABLE.DataType = 'single'
  LL_MAX_DRIVER_TORQUE_ENABLE.Dimensions = [1 1]
  LL_MAX_LANE_WIDTH_DISABLE = Simulink.Parameter
  LL_MAX_LANE_WIDTH_DISABLE.Value = 5.5
  LL_MAX_LANE_WIDTH_DISABLE.DataType = 'single'
  LL_MAX_LANE_WIDTH_DISABLE.Dimensions = [1 1]
  LL_MAX_LANE_WIDTH_ENABLE = Simulink.Parameter
  LL_MAX_LANE_WIDTH_ENABLE.Value = 5.4
  LL_MAX_LANE_WIDTH_ENABLE.DataType = 'single'
  LL_MAX_LANE_WIDTH_ENABLE.Dimensions = [1 1]
  LL_MAX_LAT_ACC_DISABLE = Simulink.Parameter
  LL_MAX_LAT_ACC_DISABLE.Value = 3.5
  LL_MAX_LAT_ACC_DISABLE.DataType = 'single'
  LL_MAX_LAT_ACC_DISABLE.Dimensions = [1 1]
  LL_MAX_LAT_ACC_ENABLE = Simulink.Parameter
  LL_MAX_LAT_ACC_ENABLE.Value = 3
  LL_MAX_LAT_ACC_ENABLE.DataType = 'single'
  LL_MAX_LAT_ACC_ENABLE.Dimensions = [1 1]
  LL_MAX_LDWS_SPEED_DISABLE = Simulink.Parameter
  LL_MAX_LDWS_SPEED_DISABLE.Value = 150
  LL_MAX_LDWS_SPEED_DISABLE.DataType = 'single'
  LL_MAX_LDWS_SPEED_DISABLE.Dimensions = [1 1]
  LL_MAX_LDWS_SPEED_ENABLE = Simulink.Parameter
  LL_MAX_LDWS_SPEED_ENABLE.Value = 140
  LL_MAX_LDWS_SPEED_ENABLE.DataType = 'single'
  LL_MAX_LDWS_SPEED_ENABLE.Dimensions = [1 1]
  LL_MAX_LKAS_SPEED_DISABLE = Simulink.Parameter
  LL_MAX_LKAS_SPEED_DISABLE.Value = 150
  LL_MAX_LKAS_SPEED_DISABLE.DataType = 'single'
  LL_MAX_LKAS_SPEED_DISABLE.Dimensions = [1 1]
  LL_MAX_LKAS_SPEED_ENABLE = Simulink.Parameter
  LL_MAX_LKAS_SPEED_ENABLE.Value = 140
  LL_MAX_LKAS_SPEED_ENABLE.DataType = 'single'
  LL_MAX_LKAS_SPEED_ENABLE.Dimensions = [1 1]
  LL_MAX_LONG_ACC_DISABLE = Simulink.Parameter
  LL_MAX_LONG_ACC_DISABLE.Value = 3.5
  LL_MAX_LONG_ACC_DISABLE.DataType = 'single'
  LL_MAX_LONG_ACC_DISABLE.Dimensions = [1 1]
  LL_MAX_LONG_ACC_ENABLE = Simulink.Parameter
  LL_MAX_LONG_ACC_ENABLE.Value = 3
  LL_MAX_LONG_ACC_ENABLE.DataType = 'single'
  LL_MAX_LONG_ACC_ENABLE.Dimensions = [1 1]
  LL_MAX_LONG_DECEL_DISABLE = Simulink.Parameter
  LL_MAX_LONG_DECEL_DISABLE.Value = 2.5
  LL_MAX_LONG_DECEL_DISABLE.DataType = 'single'
  LL_MAX_LONG_DECEL_DISABLE.Dimensions = [1 1]
  LL_MAX_LONG_DECEL_ENABLE = Simulink.Parameter
  LL_MAX_LONG_DECEL_ENABLE.Value = 2
  LL_MAX_LONG_DECEL_ENABLE.DataType = 'single'
  LL_MAX_LONG_DECEL_ENABLE.Dimensions = [1 1]
  LL_MAX_STEER_ANGLE_DISABLE = Simulink.Parameter
  LL_MAX_STEER_ANGLE_DISABLE.Value = 70
  LL_MAX_STEER_ANGLE_DISABLE.DataType = 'single'
  LL_MAX_STEER_ANGLE_DISABLE.Dimensions = [1 1]
  LL_MAX_STEER_ANGLE_ENABLE = Simulink.Parameter
  LL_MAX_STEER_ANGLE_ENABLE.Value = 60
  LL_MAX_STEER_ANGLE_ENABLE.DataType = 'single'
  LL_MAX_STEER_ANGLE_ENABLE.Dimensions = [1 1]
  LL_MAX_STEER_SPEED_DISABLE = Simulink.Parameter
  LL_MAX_STEER_SPEED_DISABLE.Value = 200
  LL_MAX_STEER_SPEED_DISABLE.DataType = 'single'
  LL_MAX_STEER_SPEED_DISABLE.Dimensions = [1 1]
  LL_MAX_STEER_SPEED_ENABLE = Simulink.Parameter
  LL_MAX_STEER_SPEED_ENABLE.Value = 180
  LL_MAX_STEER_SPEED_ENABLE.DataType = 'single'
  LL_MAX_STEER_SPEED_ENABLE.Dimensions = [1 1]
  LL_MAX_SYSTEM_CURVATURE_DISABLE = Simulink.Parameter
  LL_MAX_SYSTEM_CURVATURE_DISABLE.Value = 0.005
  LL_MAX_SYSTEM_CURVATURE_DISABLE.DataType = 'single'
  LL_MAX_SYSTEM_CURVATURE_DISABLE.Dimensions = [1 1]
  LL_MAX_SYSTEM_CURVATURE_ENABLE = Simulink.Parameter
  LL_MAX_SYSTEM_CURVATURE_ENABLE.Value = 0.004
  LL_MAX_SYSTEM_CURVATURE_ENABLE.DataType = 'single'
  LL_MAX_SYSTEM_CURVATURE_ENABLE.Dimensions = [1 1]
  LL_MIN_LANE_WIDTH_DISABLE = Simulink.Parameter
  LL_MIN_LANE_WIDTH_DISABLE.Value = 2.4
  LL_MIN_LANE_WIDTH_DISABLE.DataType = 'single'
  LL_MIN_LANE_WIDTH_DISABLE.Dimensions = [1 1]
  LL_MIN_LANE_WIDTH_ENABLE = Simulink.Parameter
  LL_MIN_LANE_WIDTH_ENABLE.Value = 2.5
  LL_MIN_LANE_WIDTH_ENABLE.DataType = 'single'
  LL_MIN_LANE_WIDTH_ENABLE.Dimensions = [1 1]
  LL_MIN_LKAS_SPEED_DISABLE = Simulink.Parameter
  LL_MIN_LKAS_SPEED_DISABLE.Value = 55
  LL_MIN_LKAS_SPEED_DISABLE.DataType = 'single'
  LL_MIN_LKAS_SPEED_DISABLE.Dimensions = [1 1]
  LL_MIN_LKAS_SPEED_ENABLE = Simulink.Parameter
  LL_MIN_LKAS_SPEED_ENABLE.Value = 60
  LL_MIN_LKAS_SPEED_ENABLE.DataType = 'single'
  LL_MIN_LKAS_SPEED_ENABLE.Dimensions = [1 1]
  LL_Max_LDWS_Warning_Time = Simulink.Parameter
  LL_Max_LDWS_Warning_Time.Value = 5
  LL_Max_LDWS_Warning_Time.DataType = 'single'
  LL_Max_LDWS_Warning_Time.Dimensions = [1 1]
  LL_NomTAhd_C = Simulink.Parameter
  LL_NomTAhd_C.Value = 0.2
  LL_NomTAhd_C.DataType = 'single'
  LL_NomTAhd_C.Dimensions = [1 1]
  LL_RlsDet_tiTDelTime_DISABLE = Simulink.Parameter
  LL_RlsDet_tiTDelTime_DISABLE.Value = 20
  LL_RlsDet_tiTDelTime_DISABLE.DataType = 'single'
  LL_RlsDet_tiTDelTime_DISABLE.Dimensions = [1 1]
  LL_RlsDet_tiTrqChkT_DISABLE = Simulink.Parameter
  LL_RlsDet_tiTrqChkT_DISABLE.Value = 0.25
  LL_RlsDet_tiTrqChkT_DISABLE.DataType = 'single'
  LL_RlsDet_tiTrqChkT_DISABLE.Dimensions = [1 1]
  LL_RlsDet_tiTrqChkT_EPS_DISABLE = Simulink.Parameter
  LL_RlsDet_tiTrqChkT_EPS_DISABLE.Value = 0.5
  LL_RlsDet_tiTrqChkT_EPS_DISABLE.DataType = 'single'
  LL_RlsDet_tiTrqChkT_EPS_DISABLE.Dimensions = [1 1]
  LL_SingleLane_Disable_Swt = Simulink.Parameter
  LL_SingleLane_Disable_Swt.Value = 1
  LL_SingleLane_Disable_Swt.DataType = 'boolean'
  LL_SingleLane_Disable_Swt.Dimensions = [1 1]
  LL_ThresDet_lDvtThresLwrLDW = Simulink.Parameter
  LL_ThresDet_lDvtThresLwrLDW.Value = 0.1
  LL_ThresDet_lDvtThresLwrLDW.DataType = 'single'
  LL_ThresDet_lDvtThresLwrLDW.Dimensions = [1 1]
  LL_ThresDet_lDvtThresLwrLKA = Simulink.Parameter
  LL_ThresDet_lDvtThresLwrLKA.Value = 0.3
  LL_ThresDet_lDvtThresLwrLKA.DataType = 'single'
  LL_ThresDet_lDvtThresLwrLKA.Dimensions = [1 1]
  LL_ThresDet_lDvtThresUprLDW = Simulink.Parameter
  LL_ThresDet_lDvtThresUprLDW.Value = 0.2
  LL_ThresDet_lDvtThresUprLDW.DataType = 'single'
  LL_ThresDet_lDvtThresUprLDW.Dimensions = [1 1]
  LL_ThresDet_lDvtThresUprLKA = Simulink.Parameter
  LL_ThresDet_lDvtThresUprLKA.Value = 0.6
  LL_ThresDet_lDvtThresUprLKA.DataType = 'single'
  LL_ThresDet_lDvtThresUprLKA.Dimensions = [1 1]
  LL_ThresDet_tiTTLCThresLDW = Simulink.Parameter
  LL_ThresDet_tiTTLCThresLDW.Value = 0.4
  LL_ThresDet_tiTTLCThresLDW.DataType = 'single'
  LL_ThresDet_tiTTLCThresLDW.Dimensions = [1 1]
  LL_ThresDet_tiTTLCThresLKA = Simulink.Parameter
  LL_ThresDet_tiTTLCThresLKA.Value = 1.5
  LL_ThresDet_tiTTLCThresLKA.DataType = 'single'
  LL_ThresDet_tiTTLCThresLKA.Dimensions = [1 1]
  LL_TkOvStChk_tiTDelTime = Simulink.Parameter
  LL_TkOvStChk_tiTDelTime.Value = 2
  LL_TkOvStChk_tiTDelTime.DataType = 'single'
  LL_TkOvStChk_tiTDelTime.Dimensions = [1 1]
  LL_TkOvStChk_tiTDelTime_DEACTV = Simulink.Parameter
  LL_TkOvStChk_tiTDelTime_DEACTV.Value = 1
  LL_TkOvStChk_tiTDelTime_DEACTV.DataType = 'single'
  LL_TkOvStChk_tiTDelTime_DEACTV.Dimensions = [1 1]
  LL_TkOvStChk_tiTrqChkT = Simulink.Parameter
  LL_TkOvStChk_tiTrqChkT.Value = 0.1
  LL_TkOvStChk_tiTrqChkT.DataType = 'single'
  LL_TkOvStChk_tiTrqChkT.Dimensions = [1 1]
  LL_TkOvStChk_tiTrqChkT_DEACTV = Simulink.Parameter
  LL_TkOvStChk_tiTrqChkT_DEACTV.Value = 0.1
  LL_TkOvStChk_tiTrqChkT_DEACTV.DataType = 'single'
  LL_TkOvStChk_tiTrqChkT_DEACTV.Dimensions = [1 1]
  LL_lStpLngth_C = Simulink.Parameter
  LL_lStpLngth_C.Value = 5
  LL_lStpLngth_C.DataType = 'single'
  LL_lStpLngth_C.Dimensions = [1 1]
undefined symbols (not defined in the file): LKA_CarWidth, LKA_SampleTime, LKA_StrRatio_C, LKA_Veh2CamL_C, LKA_Veh2CamW_C, LKA_WhlBaseL_C, LL_CompHdAg_C, LL_CompSWA_C, LL_CrvtPrvwT_C, LL_DesDvt_C, LL_DvtComp_C, LL_DvtPrvwT_C, LL_DvtSpdDet_vDvtSpdMin_C, LL_HandsOff_ExitTime, LL_HandsOff_TextTime, LL_HandsOff_WarnTime, LL_HdAgExT_C, LL_HdAgPrvwT_C, LL_LAccMax_C, LL_LAccRMax_C, LL_LDW_EarliestWarnLine_C, LL_LDW_LatestWarnLine_C, LL_LDWS_SUPPRESS_HEADING, LL_LFClb_TFC_FfCtlRatio_C, LL_LFClb_TFC_KdBalance_C, LL_LFClb_TFC_KdMaxSWA_C, LL_LFClb_TFC_KdV1_C, LL_LFClb_TFC_KdV2_C, LL_LFClb_TFC_KdVehSpdLwr_C, LL_LFClb_TFC_KdVehSpdUpr_C, LL_LFClb_TFC_Ki_C, LL_LFClb_TFC_KiMaxSWA_C, LL_LFClb_TFC_Kp_C, LL_LFClb_TFC_KpKlat_C, LL_LFClb_TFC_KpV1_C, LL_LFClb_TFC_KpV2_C, LL_LFClb_TFC_KpVehSpdLwr_C, LL_LFClb_TFC_KpVehSpdUpr_C, LL_LFClb_TFC_PrvwT_C, LL_LKA_EarliestWarnLine_C, LL_LKA_LatestWarnLine_C, LL_LKAExPrcs_ExitC0Dvt, LL_LKAExPrcs_ExitC0Swt, LL_LKAExPrcs_tiExitTime1, LL_LKAExPrcs_tiExitTime2, LL_LKAExPrcs_tiExitTime3, LL_LKAS_OUT_OF_CONTROL_LAT_VEL, LL_LKAS_OUT_OF_CONTROL_TTLC, LL_LKASWASyn_M0, LL_LKASWASyn_M1, LL_LKASWASyn_M2, LL_LKASWASyn_M3K, LL_LKASWASyn_SWAaddMax, LL_LKASWASyn_T2, LL_LKASWASyn_tiTrqSwaRtTime, LL_LKASWASyn_tiTrqSwaTime, LL_LKASWASyn_TrqMax, LL_LKASWASyn_TrqSwaAddSwt, LL_LKASWASyn_TrqSwaRateDiff, LL_LSpdCompT_C ... (+43)
libraries: simulink x138, canmsglib x8, dspstat3 x3, simulink_extras x1
PreSaveFcn:
  | try
  | a = datestr(now,'yyyymmdd');
  | set_param('LKAS/LKAS/LL/Version', 'Value', a(3:8));
  | clear a;
  | catch
  | end
settings Model: Creator=yxy91  LastModifiedBy=xiaoyang
settings OptimizationCC: BlockReduction=off  DefaultParameterBehavior=Inlined  UseDivisionForNetSlopeComputation=on  UseFloatMulNetSlope=on  DefaultUnderspecifiedDataType=single  UseSpecifiedMinMax=on  InlineInvariantSignals=on  PassReuseOutputArgsAs=Individual arguments  ZeroExternalMemoryAtStartup=off  ZeroInternalMemoryAtStartup=off  NoFixptDivByZeroProtection=on  EfficientFloat2IntCast=on  LifeSpan=inf  OptimizeBlockOrder=speed  DifferentSizesBufferReuse=on
settings DebuggingCC: SignalInfNanChecking=error  ReadBeforeWriteMsg=EnableAllAsError  WriteAfterWriteMsg=EnableAllAsError  WriteAfterReadMsg=EnableAllAsError  IntegerOverflowMsg=error  ParameterTunabilityLossMsg=error  UniqueDataStoreMsg=error  AssertControl=DisableAll  NonBusSignalsTreatedAsBus=error  SFInvalidInputDataAccessInChartInitDiag=error  SFTransitionOutsideNaturalParentDiag=error  SFUnreachableExecutionPathDiag=error  SFUndirectedBroadcastEventsDiag=error  IntegerSaturationMsg=error
settings HardwareCC: ProdLongLongMode=on
settings ModelReferenceCC: UpdateModelReferenceTargets=IfOutOfDate
settings SFSimCC: SFSimEcho=off  CompileTimeRecursionLimit=0  EnableRuntimeRecursion=off  MATLABDynamicMemAlloc=off
settings RTWCC: SystemTargetFile=autosar.tlc  GenCodeOnly=on  TemplateMakefile=ert_default_tmf  Description=AUTOSAR  GenerateReport=on  BuildConfiguration=Faster Runs  IncludeHyperlinkInReport=on  LaunchReport=on  GenerateTraceInfo=on  GenerateTraceReport=on  GenerateTraceReportSl=on  GenerateTraceReportSf=on  GenerateTraceReportEml=on  GenerateCodeMetricsReport=on  GenerateCodeReplacementReport=on
settings CodeAppCC: ForceParamTrailComments=on  IgnoreCustomStorageClasses=off  OperatorAnnotations=on  SimulinkDataObjDesc=on  SFDataObjDesc=on  MATLABFcnDesc=on  InsertBlockDesc=on  StateflowObjectComments=on  MATLABSourceComments=on  EnableCustomComments=on  ReqsInCode=on
settings STFCustomTargetCC: TargetLangStandard=C99 (ISO)  UtilityFuncGeneration=Shared location  MultiwordLength=256  ParMdlRefBuildCompliant=on  CompOptLevelCompliant=on  IncludeMdlTerminateFcn=off  CombineOutputUpdateFcns=on  CombineSignalStateStructs=on  SuppressErrorStatus=on  ERTCustomFileBanners=on  SupportNonFinite=off  SupportComplex=off  SupportContinuousTime=off  SupportNonInlinedSFcns=off  RemoveResetFunc=on  ParenthesesLevel=Maximum  CastingMode=Standards  MATLABClassNameForMDSCustomization=Simulink.SoftwareTarget.ERTCustomization  AutosarCompliant=on  UseToolchainInfoCompliant=on  GenerateSharedConstants=off  LookupTableObjectStructAxisOrder=2,1,3,4,...  LUTObjectStructOrderEvenSpacing=Size,Table,Breakpoints  SystemTargetFile=autosar.tlc
settings ERTTargetCC: TargetLangStandard=C99 (ISO)  UtilityFuncGeneration=Shared location  ConcurrentExecutionCompliant=off  IncludeMdlTerminateFcn=off  CombineSignalStateStructs=on  SuppressErrorStatus=on  SupportNonFinite=off  SupportComplex=off  ParenthesesLevel=Maximum  CastingMode=Standards  ModelStepFunctionPrototypeControlCompliant=off  CPPClassGenCompliant=off  AutosarCompliant=on  GenerateSharedConstants=off  LookupTableObjectStructAxisOrder=2,1,3,4,...  LUTObjectStructOrderEvenSpacing=Size,Table,Breakpoints  GenerateASAP2=on  InlinedParameterPlacement=NonHierarchical  ERTCustomFileTemplate=example_file_process.tlc  EnableSignedLeftShifts=off  EnableSignedRightShifts=off
settings ConfigComp: PSVerificationMode=BugFinder  PSVerificationSettings=PrjConfigAndMisraC2012  PSResultDir=D:\LKAS\bin\LKAS_CodeTest_20220118_1027  PSAutoStubLUT=on  PSEnablePrjConfigFile=on  PSPrjConfigFile=D:\LKAS\LKAS.psprj

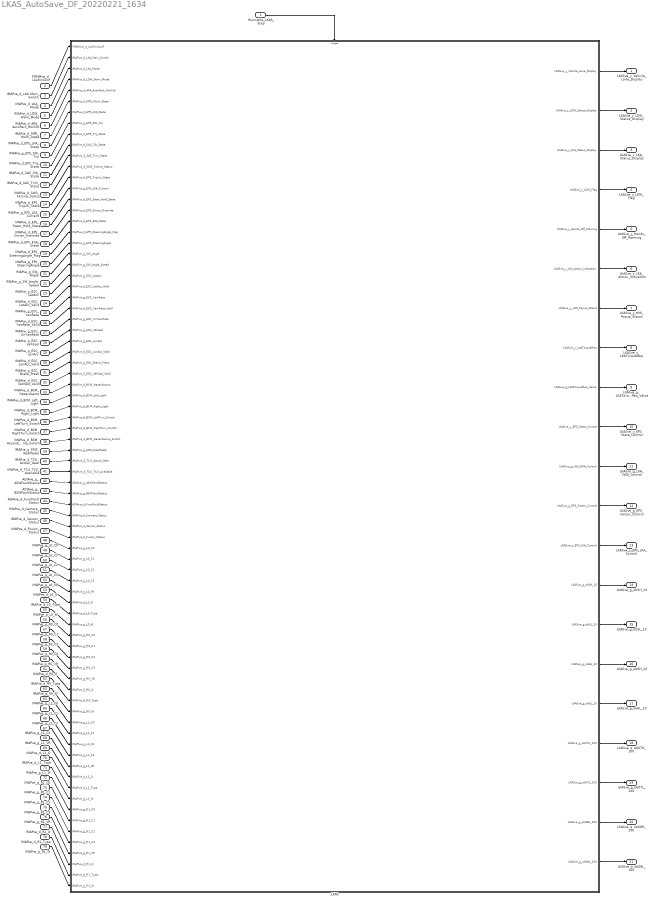
== system LKAS_AutoSave_DF_20220221_1634 ==
  Runnable_LKAS_Step : Inport  SampleTime=0.01  OutputFunctionCall=on
  FDMMve_d_LkaFcnConf : Inport  Port=2  OutDataTypeStr=UInt16  PortDimensions=1
  IMAPve_d_LKA_Main_Switch : Inport  Port=3  OutDataTypeStr=UInt16  PortDimensions=1
  IMAPve_d_LKA_Mode : Inport  Port=4  OutDataTypeStr=UInt16  PortDimensions=1
  IMAPve_d_LDW_Warn_Mode : Inport  Port=5  OutDataTypeStr=UInt16  PortDimensions=1
  IMAPve_d_APA_AutoPark_WorkSt : Inport  Port=6  OutDataTypeStr=UInt16  PortDimensions=1
  IMAPve_d_MP5_Work_State : Inport  Port=7  OutDataTypeStr=UInt16  PortDimensions=1
  IMAPve_d_EPS_LKA_State : Inport  Port=8  OutDataTypeStr=UInt16  PortDimensions=1
  IMAPve_g_EPS_SW_Trq : Inport  Port=9  OutDataTypeStr=T_M_Nm_Float32  PortDimensions=1
  IMAPve_d_EPS_Trq_State : Inport  Port=10  OutDataTypeStr=UInt16  PortDimensions=1
  IMAPve_d_SAS_Clb_State : Inport  Port=11  OutDataTypeStr=UInt16  PortDimensions=1
  IMAPve_d_SAS_Trim_State : Inport  Port=12  OutDataTypeStr=UInt16  PortDimensions=1
  IMAPve_d_SWS_Failure_Status : Inport  Port=13  OutDataTypeStr=UInt16  PortDimensions=1
  IMAPve_d_EPS_TrqLim_State : Inport  Port=14  OutDataTypeStr=UInt16  PortDimensions=1
  IMAPve_g_EPS_LKA_Current : Inport  Port=15  OutDataTypeStr=T_M_Nm_Float32  PortDimensions=1
  IMAPve_d_EPS_Steer_Hold_State : Inport  Port=16  OutDataTypeStr=UInt16  PortDimensions=1
  IMAPve_d_EPS_Driver_Override : Inport  Port=17  OutDataTypeStr=UInt16  PortDimensions=1
  IMAPve_d_EPS_ESA_State : Inport  Port=18  OutDataTypeStr=UInt16  PortDimensions=1
  IMAPve_d_EPS_SteeringAngle_Flag : Inport  Port=19  OutDataTypeStr=UInt16  PortDimensions=1
  IMAPve_g_EPS_SteeringAngle : Inport  Port=20  OutDataTypeStr=T_M_Nm_Float32  PortDimensions=1
  IMAPve_g_SW_Angle : Inport  Port=21  OutDataTypeStr=T_M_Nm_Float32  PortDimensions=1
  IMAPve_g_SW_Angle_Speed : Inport  Port=22  OutDataTypeStr=T_M_Nm_Float32  PortDimensions=1
  IMAPve_g_ESC_LatAcc : Inport  Port=23  OutDataTypeStr=T_M_Nm_Float32  PortDimensions=1
  IMAPve_d_ESC_LatAcc_Valid : Inport  Port=24  OutDataTypeStr=UInt16  PortDimensions=1
  IMAPve_g_ESC_YawRate : Inport  Port=25  OutDataTypeStr=T_M_Nm_Float32  PortDimensions=1
  IMAPve_d_ESC_YawRate_Valid : Inport  Port=26  OutDataTypeStr=UInt16  PortDimensions=1
  IMAPve_g_ESC_UnYawRate : Inport  Port=27  OutDataTypeStr=T_M_Nm_Float32  PortDimensions=1
  IMAPve_g_ESC_VehSpd : Inport  Port=28  OutDataTypeStr=T_M_Nm_Float32  PortDimensions=1
  IMAPve_g_ESC_LonAcc : Inport  Port=29  OutDataTypeStr=T_M_Nm_Float32  PortDimensions=1
  IMAPve_d_ESC_LonAcc_Valid : Inport  Port=30  OutDataTypeStr=UInt16  PortDimensions=1
  IMAPve_g_ESC_Brake_Press : Inport  Port=31  OutDataTypeStr=T_M_Nm_Float32  PortDimensions=1
  IMAPve_d_ESC_VehSpd_Valid : Inport  Port=32  OutDataTypeStr=UInt16  PortDimensions=1
  IMAPve_d_BCM_HazardLamp : Inport  Port=33  OutDataTypeStr=UInt16  PortDimensions=1
  IMAPve_d_BCM_Left_Light : Inport  Port=34  OutDataTypeStr=UInt16  PortDimensions=1
  IMAPve_d_BCM_Right_Light : Inport  Port=35  OutDataTypeStr=UInt16  PortDimensions=1
  IMAPve_d_BCM_LeftTurn_Switch : Inport  Port=36  OutDataTypeStr=UInt16  PortDimensions=1
  IMAPve_d_BCM_RightTurn_Switch : Inport  Port=37  OutDataTypeStr=UInt16  PortDimensions=1
  IMAPve_d_BCM_HazardLamp_Switch : Inport  Port=38  OutDataTypeStr=UInt16
  IMAPve_g_EMS_RealPedal : Inport  Port=39  OutDataTypeStr=T_M_Nm_Float32  PortDimensions=1
  IMAPve_d_TCU_Actual_Gear : Inport  Port=40  OutDataTypeStr=UInt16  PortDimensions=1
  IMAPve_d_TCU_TCU_Available : Inport  Port=41  OutDataTypeStr=UInt16  PortDimensions=1
  ADIAve_g_ASWFaultStatus : Inport  Port=42  OutDataTypeStr=UInt32
  ADIAve_g_BSWFaultStatus : Inport  Port=43  OutDataTypeStr=UInt32
  ADIAve_d_FuncFaultStatus : Inport  Port=44  OutDataTypeStr=UInt16
  IMAPve_d_Camera_Status : Inport  Port=45  OutDataTypeStr=UInt16  PortDimensions=1
  IMAPve_d_Sensor_Status : Inport  Port=46  OutDataTypeStr=UInt16  PortDimensions=1
  IMAPve_d_Fusion_Status : Inport  Port=47  OutDataTypeStr=UInt16  PortDimensions=1
  IMAPve_g_L0_C0 : Inport  Port=48  OutDataTypeStr=T_M_Nm_Float32  PortDimensions=1
  IMAPve_g_L0_C1 : Inport  Port=49  OutDataTypeStr=T_M_Nm_Float32  PortDimensions=1
  IMAPve_g_L0_C2 : Inport  Port=50  OutDataTypeStr=T_M_Nm_Float32  PortDimensions=1
  IMAPve_g_L0_C3 : Inport  Port=51  OutDataTypeStr=T_M_Nm_Float32  PortDimensions=1
  IMAPve_g_L0_VR : Inport  Port=52  OutDataTypeStr=T_M_Nm_Float32  PortDimensions=1
  IMAPve_d_L0_Q : Inport  Port=53  OutDataTypeStr=UInt16  PortDimensions=1
  IMAPve_d_L0_Type : Inport  Port=54  OutDataTypeStr=UInt16  PortDimensions=1
  IMAPve_g_L0_W : Inport  Port=55  OutDataTypeStr=T_M_Nm_Float32  PortDimensions=1
  IMAPve_g_R0_C0 : Inport  Port=56  OutDataTypeStr=T_M_Nm_Float32  PortDimensions=1
  IMAPve_g_R0_C1 : Inport  Port=57  OutDataTypeStr=T_M_Nm_Float32  PortDimensions=1
  IMAPve_g_R0_C2 : Inport  Port=58  OutDataTypeStr=T_M_Nm_Float32  PortDimensions=1
  IMAPve_g_R0_C3 : Inport  Port=59  OutDataTypeStr=T_M_Nm_Float32  PortDimensions=1
  IMAPve_g_R0_VR : Inport  Port=60  OutDataTypeStr=T_M_Nm_Float32  PortDimensions=1
  IMAPve_d_R0_Q : Inport  Port=61  OutDataTypeStr=UInt16  PortDimensions=1
  IMAPve_d_R0_Type : Inport  Port=62  OutDataTypeStr=UInt16  PortDimensions=1
  IMAPve_g_R0_W : Inport  Port=63  OutDataTypeStr=T_M_Nm_Float32  PortDimensions=1
  IMAPve_g_L1_C0 : Inport  Port=64  OutDataTypeStr=T_M_Nm_Float32  PortDimensions=1
  IMAPve_g_L1_C1 : Inport  Port=65  OutDataTypeStr=T_M_Nm_Float32  PortDimensions=1
  IMAPve_g_L1_C2 : Inport  Port=66  OutDataTypeStr=T_M_Nm_Float32  PortDimensions=1
  IMAPve_g_L1_C3 : Inport  Port=67  OutDataTypeStr=T_M_Nm_Float32  PortDimensions=1
  IMAPve_g_L1_VR : Inport  Port=68  OutDataTypeStr=T_M_Nm_Float32  PortDimensions=1
  IMAPve_d_L1_Q : Inport  Port=69  OutDataTypeStr=UInt16  PortDimensions=1
  IMAPve_d_L1_Type : Inport  Port=70  OutDataTypeStr=UInt16  PortDimensions=1
  IMAPve_g_L1_W : Inport  Port=71  OutDataTypeStr=T_M_Nm_Float32  PortDimensions=1
  IMAPve_g_R1_C0 : Inport  Port=72  OutDataTypeStr=T_M_Nm_Float32  PortDimensions=1
  IMAPve_g_R1_C1 : Inport  Port=73  OutDataTypeStr=T_M_Nm_Float32  PortDimensions=1
  IMAPve_g_R1_C2 : Inport  Port=74  OutDataTypeStr=T_M_Nm_Float32  PortDimensions=1
  IMAPve_g_R1_C3 : Inport  Port=75  OutDataTypeStr=T_M_Nm_Float32  PortDimensions=1
  IMAPve_g_R1_VR : Inport  Port=76  OutDataTypeStr=T_M_Nm_Float32  PortDimensions=1
  IMAPve_d_R1_Q : Inport  Port=77  OutDataTypeStr=UInt16  PortDimensions=1
  IMAPve_d_R1_Type : Inport  Port=78  OutDataTypeStr=UInt16  PortDimensions=1
  IMAPve_g_R1_W : Inport  Port=79  OutDataTypeStr=T_M_Nm_Float32  PortDimensions=1
  LKAS : Subsystem  TreatAsAtomicUnit=on
  LKASve_y_Vehicle_Lane_Display : Outport  OutDataTypeStr=UInt8  PortDimensions=1
  LKASve_y_LDW_Status_Display : Outport  Port=2  OutDataTypeStr=UInt8  PortDimensions=1
  LKASve_y_LKA_Status_Display : Outport  Port=3  OutDataTypeStr=UInt8  PortDimensions=1
  LKASve_y_LDW_Flag : Outport  Port=4  OutDataTypeStr=UInt8  PortDimensions=1
  LKASve_y_Hands_Off_Warning : Outport  Port=5  OutDataTypeStr=UInt8  PortDimensions=1
  LKASve_y_LKA_Action_Indication : Outport  Port=6  OutDataTypeStr=UInt8  PortDimensions=1
  LKASve_y_HMI_Popup_Status : Outport  Port=7  OutDataTypeStr=UInt8  PortDimensions=1
  LKASve_y_LKATorqueReq : Outport  Port=8  OutDataTypeStr=UInt8  PortDimensions=1
  LKASve_g_LKATorqueReq_Value : Outport  Port=9  OutDataTypeStr=T_M_Nm_Float32  PortDimensions=1
  LKASve_y_EPS_State_Control : Outport  Port=10  OutDataTypeStr=UInt8  PortDimensions=1
  LKASve_g_LKA_SWA_Control : Outport  Port=11  OutDataTypeStr=T_M_Nm_Float32  PortDimensions=1
  LKASve_g_EPS_Factor_Control : Outport  Port=12  OutDataTypeStr=T_M_Nm_Float32  PortDimensions=1
  LKASve_y_EPS_LKA_Control : Outport  Port=13  OutDataTypeStr=UInt8  PortDimensions=1
  LKASve_g_ob5H_10 : Outport  Port=14  OutDataTypeStr=UInt32  PortDimensions=1
  LKASve_g_ob5L_10 : Outport  Port=15  OutDataTypeStr=UInt32  PortDimensions=1
  LKASve_g_ob6H_10 : Outport  Port=16  OutDataTypeStr=UInt32  PortDimensions=1
  LKASve_g_ob6L_10 : Outport  Port=17  OutDataTypeStr=UInt32  PortDimensions=1
  LKASve_g_ob07H_100 : Outport  Port=18  OutDataTypeStr=UInt32  PortDimensions=1
  LKASve_g_ob07L_100 : Outport  Port=19  OutDataTypeStr=UInt32  PortDimensions=1
  LKASve_g_ob08H_100 : Outport  Port=20  OutDataTypeStr=UInt32  PortDimensions=1
  LKASve_g_ob08L_100 : Outport  Port=21  OutDataTypeStr=UInt32  PortDimensions=1
  wires:
  FDMMve_d_LkaFcnConf/1 -> LKAS/1(FDMMve_d_LkaFcnConf)
  IMAPve_d_LKA_Main_Switch/1 -> LKAS/2(IMAPve_d_LKA_Main_Switch)
  IMAPve_d_LKA_Mode/1 -> LKAS/3(IMAPve_d_LKA_Mode)
  IMAPve_d_LDW_Warn_Mode/1 -> LKAS/4(IMAPve_d_LDW_Warn_Mode)
  IMAPve_d_APA_AutoPark_WorkSt/1 -> LKAS/5(IMAPve_d_APA_AutoPark_WorkSt)
  IMAPve_d_MP5_Work_State/1 -> LKAS/6(IMAPve_d_MP5_Work_State)
  IMAPve_d_EPS_LKA_State/1 -> LKAS/7(IMAPve_d_EPS_LKA_State)
  IMAPve_g_EPS_SW_Trq/1 -> LKAS/8(IMAPve_g_EPS_SW_Trq)
  IMAPve_d_EPS_Trq_State/1 -> LKAS/9(IMAPve_d_EPS_Trq_State)
  IMAPve_d_SAS_Clb_State/1 -> LKAS/10(IMAPve_d_SAS_Clb_State)
  IMAPve_d_SAS_Trim_State/1 -> LKAS/11(IMAPve_d_SAS_Trim_State)
  IMAPve_d_SWS_Failure_Status/1 -> LKAS/12(IMAPve_d_SWS_Failure_Status)
  IMAPve_d_EPS_TrqLim_State/1 -> LKAS/13(IMAPve_d_EPS_TrqLim_State)
  IMAPve_g_EPS_LKA_Current/1 -> LKAS/14(IMAPve_g_EPS_LKA_Current)
  IMAPve_d_EPS_Steer_Hold_State/1 -> LKAS/15(IMAPve_d_EPS_Steer_Hold_State)
  IMAPve_d_EPS_Driver_Override/1 -> LKAS/16(IMAPve_d_EPS_Driver_Override)
  IMAPve_d_EPS_ESA_State/1 -> LKAS/17(IMAPve_d_EPS_ESA_State)
  IMAPve_d_EPS_SteeringAngle_Flag/1 -> LKAS/18(IMAPve_d_EPS_SteeringAngle_Flag)
  IMAPve_g_EPS_SteeringAngle/1 -> LKAS/19(IMAPve_g_EPS_SteeringAngle)
  IMAPve_g_SW_Angle/1 -> LKAS/20(IMAPve_g_SW_Angle)
  IMAPve_g_SW_Angle_Speed/1 -> LKAS/21(IMAPve_g_SW_Angle_Speed)
  IMAPve_g_ESC_LatAcc/1 -> LKAS/22(IMAPve_g_ESC_LatAcc)
  IMAPve_d_ESC_LatAcc_Valid/1 -> LKAS/23(IMAPve_d_ESC_LatAcc_Valid)
  IMAPve_g_ESC_YawRate/1 -> LKAS/24(IMAPve_g_ESC_YawRate)
  IMAPve_d_ESC_YawRate_Valid/1 -> LKAS/25(IMAPve_d_ESC_YawRate_Valid)
  IMAPve_g_ESC_UnYawRate/1 -> LKAS/26(IMAPve_g_ESC_UnYawRate)
  IMAPve_g_ESC_VehSpd/1 -> LKAS/27(IMAPve_g_ESC_VehSpd)
  IMAPve_g_ESC_LonAcc/1 -> LKAS/28(IMAPve_g_ESC_LonAcc)
  IMAPve_d_ESC_LonAcc_Valid/1 -> LKAS/29(IMAPve_d_ESC_LonAcc_Valid)
  IMAPve_g_ESC_Brake_Press/1 -> LKAS/30(IMAPve_g_ESC_Brake_Press)
  IMAPve_d_ESC_VehSpd_Valid/1 -> LKAS/31(IMAPve_d_ESC_VehSpd_Valid)
  IMAPve_d_BCM_HazardLamp/1 -> LKAS/32(IMAPve_d_BCM_HazardLamp)
  IMAPve_d_BCM_Left_Light/1 -> LKAS/33(IMAPve_d_BCM_Left_Light)
  IMAPve_d_BCM_Right_Light/1 -> LKAS/34(IMAPve_d_BCM_Right_Light)
  IMAPve_d_BCM_LeftTurn_Switch/1 -> LKAS/35(IMAPve_d_BCM_LeftTurn_Switch)
  IMAPve_d_BCM_RightTurn_Switch/1 -> LKAS/36(IMAPve_d_BCM_RightTurn_Switch)
  IMAPve_g_EMS_RealPedal/1 -> LKAS/38(IMAPve_g_EMS_RealPedal)
  IMAPve_d_TCU_Actual_Gear/1 -> LKAS/39(IMAPve_d_TCU_Actual_Gear)
  IMAPve_d_TCU_TCU_Available/1 -> LKAS/40(IMAPve_d_TCU_TCU_Available)
  IMAPve_d_Camera_Status/1 -> LKAS/44(IMAPve_d_Camera_Status)
  IMAPve_d_Sensor_Status/1 -> LKAS/45(IMAPve_d_Sensor_Status)
  IMAPve_d_Fusion_Status/1 -> LKAS/46(IMAPve_d_Fusion_Status)
  IMAPve_g_L0_C0/1 -> LKAS/47(IMAPve_g_L0_C0)
  IMAPve_g_L0_C1/1 -> LKAS/48(IMAPve_g_L0_C1)
  IMAPve_g_L0_C2/1 -> LKAS/49(IMAPve_g_L0_C2)
  IMAPve_g_L0_C3/1 -> LKAS/50(IMAPve_g_L0_C3)
  IMAPve_g_L0_VR/1 -> LKAS/51(IMAPve_g_L0_VR)
  IMAPve_d_L0_Q/1 -> LKAS/52(IMAPve_d_L0_Q)
  IMAPve_d_L0_Type/1 -> LKAS/53(IMAPve_d_L0_Type)
  IMAPve_g_L0_W/1 -> LKAS/54(IMAPve_g_L0_W)
  IMAPve_g_R0_C0/1 -> LKAS/55(IMAPve_g_R0_C0)
  IMAPve_g_R0_C1/1 -> LKAS/56(IMAPve_g_R0_C1)
  IMAPve_g_R0_C2/1 -> LKAS/57(IMAPve_g_R0_C2)
  IMAPve_g_R0_C3/1 -> LKAS/58(IMAPve_g_R0_C3)
  IMAPve_g_R0_VR/1 -> LKAS/59(IMAPve_g_R0_VR)
  IMAPve_d_R0_Q/1 -> LKAS/60(IMAPve_d_R0_Q)
  IMAPve_d_R0_Type/1 -> LKAS/61(IMAPve_d_R0_Type)
  IMAPve_g_R0_W/1 -> LKAS/62(IMAPve_g_R0_W)
  IMAPve_g_L1_C0/1 -> LKAS/63(IMAPve_g_L1_C0)
  IMAPve_g_L1_C1/1 -> LKAS/64(IMAPve_g_L1_C1)
  IMAPve_g_L1_C2/1 -> LKAS/65(IMAPve_g_L1_C2)
  IMAPve_g_L1_C3/1 -> LKAS/66(IMAPve_g_L1_C3)
  IMAPve_g_L1_VR/1 -> LKAS/67(IMAPve_g_L1_VR)
  IMAPve_d_L1_Q/1 -> LKAS/68(IMAPve_d_L1_Q)
  IMAPve_d_L1_Type/1 -> LKAS/69(IMAPve_d_L1_Type)
  IMAPve_g_L1_W/1 -> LKAS/70(IMAPve_g_L1_W)
  IMAPve_g_R1_C0/1 -> LKAS/71(IMAPve_g_R1_C0)
  IMAPve_g_R1_C1/1 -> LKAS/72(IMAPve_g_R1_C1)
  IMAPve_g_R1_C2/1 -> LKAS/73(IMAPve_g_R1_C2)
  IMAPve_g_R1_C3/1 -> LKAS/74(IMAPve_g_R1_C3)
  IMAPve_g_R1_VR/1 -> LKAS/75(IMAPve_g_R1_VR)
  IMAPve_d_R1_Q/1 -> LKAS/76(IMAPve_d_R1_Q)
  IMAPve_d_R1_Type/1 -> LKAS/77(IMAPve_d_R1_Type)
  IMAPve_g_R1_W/1 -> LKAS/78(IMAPve_g_R1_W)
  Runnable_LKAS_Step/1 -> LKAS/Trigger
  LKAS/1(LKASve_y_Vehicle_Lane_Display) -> LKASve_y_Vehicle_Lane_Display/1
  LKAS/2(LKASve_y_LDW_Status_Display) -> LKASve_y_LDW_Status_Display/1
  LKAS/3(LKASve_y_LKA_Status_Display) -> LKASve_y_LKA_Status_Display/1
  LKAS/4(LKASve_y_LDW_Flag) -> LKASve_y_LDW_Flag/1
  LKAS/5(LKASve_y_Hands_Off_Warning) -> LKASve_y_Hands_Off_Warning/1
  LKAS/6(LKASve_y_LKA_Action_Indication) -> LKASve_y_LKA_Action_Indication/1
  LKAS/7(LKASve_y_HMI_Popup_Status) -> LKASve_y_HMI_Popup_Status/1
  LKAS/8(LKASve_y_LKATorqueReq) -> LKASve_y_LKATorqueReq/1
  LKAS/9(LKASve_g_LKATorqueReq_Value) -> LKASve_g_LKATorqueReq_Value/1
  LKAS/10(LKASve_y_EPS_State_Control) -> LKASve_y_EPS_State_Control/1
  LKAS/11(LKASve_g_LKA_SWA_Control) -> LKASve_g_LKA_SWA_Control/1
  LKAS/12(LKASve_g_EPS_Factor_Control) -> LKASve_g_EPS_Factor_Control/1
  LKAS/13(LKASve_y_EPS_LKA_Control) -> LKASve_y_EPS_LKA_Control/1
  LKAS/14(LKASve_g_ob5H_10) -> LKASve_g_ob5H_10/1
  LKAS/15(LKASve_g_ob5L_10) -> LKASve_g_ob5L_10/1
  LKAS/16(LKASve_g_ob6H_10) -> LKASve_g_ob6H_10/1
  LKAS/17(LKASve_g_ob6L_10) -> LKASve_g_ob6L_10/1
  LKAS/18(LKASve_g_ob07H_100) -> LKASve_g_ob07H_100/1
  LKAS/19(LKASve_g_ob07L_100) -> LKASve_g_ob07L_100/1
  LKAS/20(LKASve_g_ob08H_100) -> LKASve_g_ob08H_100/1
  LKAS/21(LKASve_g_ob08L_100) -> LKASve_g_ob08L_100/1
  ADIAve_g_ASWFaultStatus/1 -> LKAS/41(ADIAve_g_ASWFaultStatus)
  ADIAve_g_BSWFaultStatus/1 -> LKAS/42(ADIAve_g_BSWFaultStatus)
  ADIAve_d_FuncFaultStatus/1 -> LKAS/43(ADIAve_d_FuncFaultStatus)
  IMAPve_d_BCM_HazardLamp_Switch/1 -> LKAS/37(IMAPve_d_BCM_HazardLamp_Switch)
